simulink model "tracking_model"  (R2017a)
(part 9 of 14)

s(x_3).^4.*3.79080679921875e-6+sin(x_3).^4.*3.79080679921875e-6+cos(x_3).^4.*cos(x_4).^2.*6.757062187003037e-11+cos(x_3).^4.*cos(x_5).^2.*6.757062187003037e-11+cos(x_3).^4.*cos(x_6).^2.*6.757062187003037e-11+cos(x_3).^2.*sin(x_3).^2.*7.5816135984375e-6+cos(x_4).^2.*sin(x_3).^4.*6.757062187003037e-11+cos(x_5).^2.*sin(x_3).^4.*6.757062187003037e-11+cos(x_6).^2.*sin(x_3).^4.*6.757062187003037e-11+cos(x_3).^2.*cos(x_4).^2.*sin(x_3).^2.*1.351412437400607e-10+cos(x_3).^2.*cos(x_5).^2.*sin(x_3).^2.*1.351412437400607e-10+cos(x_3).^2.*cos(x_6).^2.*sin(x_3).^2.*1.351412437400607e-10)+(x_8.*x_9.*cos(x_3).^4.*cos(x_6).*sin(x_3).*sin(x_4).^4.*sin(x_6).*1.134624119983866e-24)./(cos(x_3).^4.*3.79080679921875e-6+sin(x_3).^4.*3.79080679921875e-6+cos(x_3).^4.*cos(x_4).^2.*6.757062187003037e-11+cos(x_3).^4.*cos(x_5).^2.*6.757062187003037e-11+cos(x_3).^4.*cos(x_6).^2.*6.757062187003037e-11+cos(x_3).^2.*sin(x_3).^2.*7.5816135984375e-6+cos(x_4).^2.*sin(x_3).^4.*6.757062187003037e-11+cos(x_5).^2.*sin(x_3).^4.*6.757062187003037e-11+cos(x_6).^2.*sin(x_3).^4.*6.757062187003037e-11+cos(x_3).^2.*cos(x_4).^2.*sin(x_3).^2.*1.351412437400607e-10+cos(x_3).^2.*cos(x_5).^2.*sin(x_3).^2.*1.351412437400607e-10+cos(x_3).^2.*cos(x_6).^2.*sin(x_3).^2.*1.351412437400607e-10)-(x_8.*x_9.*cos(x_3).*cos(x_6).*sin(x_3).^4.*sin(x_5).^4.*sin(x_6).*6.550755411017271e-25)./(cos(x_3).^4.*3.79080679921875e-6+sin(x_3).^4.*3.79080679921875e-6+cos(x_3).^4.*cos(x_4).^2.*6.757062187003037e-11+cos(x_3).^4.*cos(x_5).^2.*6.757062187003037e-11+cos(x_3).^4.*cos(x_6).^2.*6.757062187003037e-11+cos(x_3).^2.*sin(x_3).^2.*7.5816135984375e-6+cos(x_4).^2.*sin(x_3).^4.*6.757062187003037e-11+cos(x_5).^2.*sin(x_3).^4.*6.757062187003037e-11+cos(x_6).^2.*sin(x_3).^4.*6.757062187003037e-11+cos(x_3).^2.*cos(x_4).^2.*sin(x_3).^2.*1.351412437400607e-10+cos(x_3).^2.*cos(x_5).^2.*sin(x_3).^2.*1.351412437400607e-10+cos(x_3).^2.*cos(x_6).^2.*sin(x_3).^2.*1.351412437400607e-10)+(x_8.*x_9.*cos(x_3).^4.*cos(x_6).*sin(x_3).*sin(x_5).^4.*sin(x_6).*1.134624119983866e-24)./(cos(x_3).^4.*3.79080679921875e-6+sin(x_3).^4.*3.79080679921875e-6+cos(x_3).^4.*cos(x_4).^2.*6.757062187003037e-11+cos(x_3).^4.*cos(x_5).^2.*6.757062187003037e-11+cos(x_3).^4.*cos(x_6).^2.*6.757062187003037e-11+cos(x_3).^2.*sin(x_3).^2.*7.5816135984375e-6+cos(x_4).^2.*sin(x_3).^4.*6.757062187003037e-11+cos(x_5).^2.*sin(x_3).^4.*6.757062187003037e-11+cos(x_6).^2.*sin(x_3).^4.*6.757062187003037e-11+cos(x_3).^2.*cos(x_4).^2.*sin(x_3).^2.*1.351412437400607e-10+cos(x_3).^2.*cos(x_5).^2.*sin(x_3).^2.*1.351412437400607e-10+cos(x_3).^2.*cos(x_6).^2.*sin(x_3).^2.*1.351412437400607e-10)-(x_7.*x_9.*cos(x_3).*cos(x_4).*sin(x_3).^3.*sin(x_4).*sin(x_5).^2.*5.998516123203674e-18)./(cos(x_3).^4.*1.5163227196875e-5+sin(x_3).^4.*1.5163227196875e-5+cos(x_3).^4.*cos(x_4).^2.*2.702824874801215e-10+cos(x_3).^4.*cos(x_5).^2.*2.702824874801215e-10+cos(x_3).^4.*cos(x_6).^2.*2.702824874801215e-10+cos(x_3).^2.*sin(x_3).^2.*3.032645439375e-5+cos(x_4).^2.*sin(x_3).^4.*2.702824874801215e-10+cos(x_5).^2.*sin(x_3).^4.*2.702824874801215e-10+cos(x_6).^2.*sin(x_3).^4.*2.702824874801215e-10+cos(x_3).^2.*cos(x_4).^2.*sin(x_3).^2.*5.40564974960243e-10+cos(x_3).^2.*cos(x_5).^2.*sin(x_3).^2.*5.40564974960243e-10+cos(x_3).^2.*cos(x_6).^2.*sin(x_3).^2.*5.40564974960243e-10)-(x_7.*x_9.*cos(x_3).^3.*cos(x_4).*sin(x_3).*sin(x_4).*sin(x_5).^2.*5.998516123203674e-18)./(cos(x_3).^4.*1.5163227196875e-5+sin(x_3).^4.*1.5163227196875e-5+cos(x_3).^4.*cos(x_4).^2.*2.702824874801215e-10+cos(x_3).^4.*cos(x_5).^2.*2.702824874801215e-10+cos(x_3).^4.*cos(x_6).^2.*2.702824874801215e-10+cos(x_3).^2.*sin(x_3).^2.*3.032645439375e-5+cos(x_4).^2.*sin(x_3).^4.*2.702824874801215e-10+cos(x_5).^2.*sin(x_3).^4.*2.702824874801215e-10+cos(x_6).^2.*sin(x_3).^4.*2.702824874801215e-10+cos(x_3).^2.*cos(x_4).^2.*sin(x_3).^2.*5.40564974960243e-10+cos(x_3).^2.*cos(x_5).^2.*sin(x_3).^2.*5.40564974960243e-10+cos(x_3).^2.*cos(x_6).^2.*sin(x_3).^2.*5.40564974960243e-10)-(x_7.*x_9.*cos(x_3).*cos(x_4).*sin(x_3).^3.*sin(x_4).*sin(x_6).^2.*5.998516123203674e-18)./(cos(x_3).^4.*1.5163227196875e-5+sin(x_3).^4.*1.5163227196875e-5+cos(x_3).^4.*cos(x_4).^2.*2.702824874801215e-10+cos(x_3).^4.*cos(x_5).^2.*2.702824874801215e-10+cos(x_3).^4.*cos(x_6).^2.*2.702824874801215e-10+cos(x_3).^2.*sin(x_3).^2.*3.032645439375e-5+cos(x_4).^2.*sin(x_3).^4.*2.702824874801215e-10+cos(x_5).^2.*sin(x_3).^4.*2.702824874801215e-10+cos(x_6).^2.*sin(x_3).^4.*2.702824874801215e-10+cos(x_3).^2.*cos(x_4).^2.*sin(x_3).^2.*5.40564974960243e-10+cos(x_3).^2.*cos(x_5).^2.*sin(x_3).^2.*5.40564974960243e-10+cos(x_3).^2.*cos(x_6).^2.*sin(x_3).^2.*5.40564974960243e-10)+(x_7.*x_9.*cos(x_3).*cos(x_5).*sin(x_3).^3.*sin(x_4).^2.*sin(x_5).*1.607297550997493e-18)./(cos(x_3).^4.*1.5163227196875e-5+sin(x_3).^4.*1.5163227196875e-5+cos(x_3).^4.*cos(x_4).^2.*2.702824874801215e-10+cos(x_3).^4.*cos(x_5).^2.*2.702824874801215e-10+cos(x_3).^4.*cos(x_6).^2.*2.702824874801215e-10+cos(x_3).^2.*sin(x_3).^2.*3.032645439375e-5+cos(x_4).^2.*sin(x_3).^4.*2.702824874801215e-10+cos(x_5).^2.*sin(x_3).^4.*2.702824874801215e-10+cos(x_6).^2.*sin(x_3).^4.*2.702824874801215e-10+cos(x_3).^2.*cos(x_4).^2.*sin(x_3).^2.*5.40564974960243e-10+cos(x_3).^2.*cos(x_5).^2.*sin(x_3).^2.*5.40564974960243e-10+cos(x_3).^2.*cos(x_6).^2.*sin(x_3).^2.*5.40564974960243e-10)-(x_7.*x_9.*cos(x_3).^3.*cos(x_4).*sin(x_3).*sin(x_4).*sin(x_6).^2.*5.998516123203674e-18)./(cos(x_3).^4.*1.5163227196875e-5+sin(x_3).^4.*1.5163227196875e-5+cos(x_3).^4.*cos(x_4).^2.*2.702824874801215e-10+cos(x_3).^4.*cos(x_5).^2.*2.702824874801215e-10+cos(x_3).^4.*cos(x_6).^2.*2.702824874801215e-10+cos(x_3).^2.*sin(x_3).^2.*3.032645439375e-5+cos(x_4).^2.*sin(x_3).^4.*2.702824874801215e-10+cos(x_5).^2.*sin(x_3).^4.*2.702824874801215e-10+cos(x_6).^2.*sin(x_3).^4.*2.702824874801215e-10+cos(x_3).^2.*cos(x_4).^2.*sin(x_3).^2.*5.40564974960243e-10+cos(x_3).^2.*cos(x_5).^2.*sin(x_3).^2.*5.40564974960243e-10+cos(x_3).^2.*cos(x_6).^2.*sin(x_3).^2.*5.40564974960243e-10)+(x_7.*x_9.*cos(x_3).^3.*cos(x_5).*sin(x_3).*sin(x_4).^2.*sin(x_5).*1.607297550997493e-18)./(cos(x_3).^4.*1.5163227196875e-5+sin(x_3).^4.*1.5163227196875e-5+cos(x_3).^4.*cos(x_4).^2.*2.702824874801215e-10+cos(x_3).^4.*cos(x_5).^2.*2.702824874801215e-10+cos(x_3).^4.*cos(x_6).^2.*2.702824874801215e-10+cos(x_3).^2.*sin(x_3).^2.*3.032645439375e-5+cos(x_4).^2.*sin(x_3).^4.*2.702824874801215e-10+cos(x_5).^2.*sin(x_3).^4.*2.702824874801215e-10+cos(x_6).^2.*sin(x_3).^4.*2.702824874801215e-10+cos(x_3).^2.*cos(x_4).^2.*sin(x_3).^2.*5.40564974960243e-10+cos(x_3).^2.*cos(x_5).^2.*sin(x_3).^2.*5.40564974960243e-10+cos(x_3).^2.*cos(x_6).^2.*sin(x_3).^2.*5.40564974960243e-10)+(x_8.*x_9.*cos(x_3).*cos(x_4).*sin(x_3).^3.*sin(x_4).*sin(x_5).^2.*1.607297550997493e-18)./(cos(x_3).^4.*1.5163227196875e-5+sin(x_3).^4.*1.5163227196875e-5+cos(x_3).^4.*cos(x_4).^2.*2.702824874801215e-10+cos(x_3).^4.*cos(x_5).^2.*2.702824874801215e-10+cos(x_3).^4.*cos(x_6).^2.*2.702824874801215e-10+cos(x_3).^2.*sin(x_3).^2.*3.032645439375e-5+cos(x_4).^2.*sin(x_3).^4.*2.702824874801215e-10+cos(x_5).^2.*sin(x_3).^4.*2.702824874801215e-10+cos(x_6).^2.*sin(x_3).^4.*2.702824874801215e-10+cos(x_3).^2.*cos(x_4).^2.*sin(x_3).^2.*5.40564974960243e-10+cos(x_3).^2.*cos(x_5).^2.*sin(x_3).^2.*5.40564974960243e-10+cos(x_3).^2.*cos(x_6).^2.*sin(x_3).^2.*5.40564974960243e-10)+(x_8.*x_9.*cos(x_3).^3.*cos(x_4).*sin(x_3).*sin(x_4).*sin(x_5).^2.*1.607297550997493e-18)./(cos(x_3).^4.*1.5163227196875e-5+sin(x_3).^4.*1.5163227196875e-5+cos(x_3).^4.*cos(x_4).^2.*2.702824874801215e-10+cos(x_3).^4.*cos(x_5).^2.*2.702824874801215e-10+cos(x_3).^4.*cos(x_6).^2.*2.702824874801215e-10+cos(x_3).^2.*sin(x_3).^2.*3.032645439375e-5+cos(x_4).^2.*sin(x_3).^4.*2.702824874801215e-10+cos(x_5).^2.*sin(x_3).^4.*2.702824874801215e-10+cos(x_6).^2.*sin(x_3).^4.*2.702824874801215e-10+cos(x_3).^2.*cos(x_4).^2.*sin(x_3).^2.*5.40564974960243e-10+cos(x_3).^2.*cos(x_5).^2.*sin(x_3).^2.*5.40564974960243e-10+cos(x_3).^2.*cos(x_6).^2.*sin(x_3).^2.*5.40564974960243e-10)+(x_8.*x_9.*cos(x_3).*cos(x_4).*sin(x_3).^3.*sin(x_4).*sin(x_6).^2.*1.607297550997493e-18)./(cos(x_3).^4.*1.5163227196875e-5+sin(x_3).^4.*1.5163227196875e-5+cos(x_3).^4.*cos(x_4).^2.*2.702824874801215e-10+cos(x_3).^4.*cos(x_5).^2.*2.702824874801215e-10+cos(x_3).^4.*cos(x_6).^2.*2.702824874801215e-10+cos(x_3).^2.*sin(x_3).^2.*3.032645439375e-5+cos(x_4).^2.*sin(x_3).^4.*2.702824874801215e-10+cos(x_5).^2.*sin(x_3).^4.*2.702824874801215e-10+cos(x_6).^2.*sin(x_3).^4.*2.702824874801215e-10+cos(x_3).^2.*cos(x_4).^2.*sin(x_3).^2.*5.40564974960243e-10+cos(x_3).^2.*cos(x_5).^2.*sin(x_3).^2.*5.40564974960243e-10+cos(x_3).^2.*cos(x_6).^2.*sin(x_3).^2.*5.40564974960243e-10)-(x_8.*x_9.*cos(x_3).*cos(x_5).*sin(x_3).^3.*sin(x_4).^2.*sin(x_5).*5.998516123203674e-18)./(cos(x_3).^4.*1.5163227196875e-5+sin(x_3).^4.*1.5163227196875e-5+cos(x_3).^4.*cos(x_4).^2.*2.702824874801215e-10+cos(x_3).^4.*cos(x_5).^2.*2.702824874801215e-10+cos(x_3).^4.*cos(x_6).^2.*2.702824874801215e-10+cos(x_3).^2.*sin(x_3).^2.*3.032645439375e-5+cos(x_4).^2.*sin(x_3).^4.*2.702824874801215e-10+cos(x_5).^2.*sin(x_3).^4.*2.702824874801215e-10+cos(x_6).^2.*sin(x_3).^4.*2.702824874801215e-10+cos(x_3).^2.*cos(x_4).^2.*sin(x_3).^2.*5.40564974960243e-10+cos(x_3).^2.*cos(x_5).^2.*sin(x_3).^2.*5.40564974960243e-10+cos(x_3).^2.*cos(x_6).^2.*sin(x_3).^2.*5.40564974960243e-10)+(x_8.*x_9.*cos(x_3).^3.*cos(x_4).*sin(x_3).*sin(x_4).*sin(x_6).^2.*1.607297550997493e-18)./(cos(x_3).^4.*1.5163227196875e-5+sin(x_3).^4.*1.5163227196875e-5+cos(x_3).^4.*cos(x_4).^2.*2.702824874801215e-10+cos(x_3).^4.*cos(x_5).^2.*2.702824874801215e-10+cos(x_3).^4.*cos(x_6).^2.*2.702824874801215e-10+cos(x_3).^2.*sin(x_3).^2.*3.032645439375e-5+cos(x_4).^2.*sin(x_3).^4.*2.702824874801215e-10+cos(x_5).^2.*sin(x_3).^4.*2.702824874801215e-10+cos(x_6).^2.*sin(x_3).^4.*2.702824874801215e-10+cos(x_3).^2.*cos(x_4).^2.*sin(x_3).^2.*5.40564974960243e-10+cos(x_3).^2.*cos(x_5).^2.*sin(x_3).^2.*5.40564974960243e-10+cos(x_3).^2.*cos(x_6).^2.*sin(x_3).^2.*5.40564974960243e-10)-(x_8.*x_9.*cos(x_3).^3.*cos(x_5).*sin(x_3).*sin(x_4).^2.*sin(x_5).*5.998516123203674e-18)./(cos(x_3).^4.*1.5163227196875e-5+sin(x_3).^4.*1.5163227196875e-5+cos(x_3).^4.*cos(x_4).^2.*2.702824874801215e-10+cos(x_3).^4.*cos(x_5).^2.*2.702824874801215e-10+cos(x_3).^4.*cos(x_6).^2.*2.702824874801215e-10+cos(x_3).^2.*sin(x_3).^2.*3.032645439375e-5+cos(x_4).^2.*sin(x_3).^4.*2.702824874801215e-10+cos(x_5).^2.*sin(x_3).^4.*2.702824874801215e-10+cos(x_6).^2.*sin(x_3).^4.*2.702824874801215e-10+cos(x_3).^2.*cos(x_4).^2.*sin(x_3).^2.*5.40564974960243e-10+cos(x_3).^2.*cos(x_5).^2.*sin(x_3).^2.*5.40564974960243e-10+cos(x_3).^2.*cos(x_6).^2.*sin(x_3).^2.*5.40564974960243e-10)+(x_7.*x_9.*cos(x_3).*cos(x_5).*sin(x_3).^3.*sin(x_5).*sin(x_6).^2.*1.607297550997493e-18)./(cos(x_3).^4.*1.5163227196875e-5+sin(x_3).^4.*1.5163227196875e-5+cos(x_3).^4.*cos(x_4).^2.*2.702824874801215e-10+cos(x_3).^4.*cos(x_5).^2.*2.702824874801215e-10+cos(x_3).^4.*cos(x_6).^2.*2.702824874801215e-10+cos(x_3).^2.*sin(x_3).^2.*3.032645439375e-5+cos(x_4).^2.*sin(x_3).^4.*2.702824874801215e-10+cos(x_5).^2.*sin(x_3).^4.*2.702824874801215e-10+cos(x_6).^2.*sin(x_3).^4.*2.702824874801215e-10+cos(x_3).^2.*cos(x_4).^2.*sin(x_3).^2.*5.40564974960243e-10+cos(x_3).^2.*cos(x_5).^2.*sin(x_3).^2.*5.40564974960243e-10+cos(x_3).^2.*cos(x_6).^2.*sin(x_3).^2.*5.40564974960243e-10)+(x_7.*x_9.*cos(x_3).*cos(x_6).*sin(x_3).^3.*sin(x_4).^2.*sin(x_6).*4.39121857220618e-18)./(cos(x_3).^4.*1.5163227196875e-5+sin(x_3).^4.*1.5163227196875e-5+cos(x_3).^4.*cos(x_4).^2.*2.702824874801215e-10+cos(x_3).^4.*cos(x_5).^2.*2.702824874801215e-10+cos(x_3).^4.*cos(x_6).^2.*2.702824874801215e-10+cos(x_3).^2.*sin(x_3).^2.*3.032645439375e-5+cos(x_4).^2.*sin(x_3).^4.*2.702824874801215e-10+cos(x_5).^2.*sin(x_3).^4.*2.702824874801215e-10+cos(x_6).^2.*sin(x_3).^4.*2.702824874801215e-10+cos(x_3).^2.*cos(x_4).^2.*sin(x_3).^2.*5.40564974960243e-10+cos(x_3).^2.*cos(x_5).^2.*sin(x_3).^2.*5.40564974960243e-10+cos(x_3).^2.*cos(x_6).^2.*sin(x_3).^2.*5.40564974960243e-10)+(x_7.*x_9.*cos(x_3).^3.*cos(x_5).*sin(x_3).*sin(x_5).*sin(x_6).^2.*1.607297550997493e-18)./(cos(x_3).^4.*1.5163227196875e-5+sin(x_3).^4.*1.5163227196875e-5+cos(x_3).^4.*cos(x_4).^2.*2.702824874801215e-10+cos(x_3).^4.*cos(x_5).^2.*2.702824874801215e-10+cos(x_3).^4.*cos(x_6).^2.*2.702824874801215e-10+cos(x_3).^2.*sin(x_3).^2.*3.032645439375e-5+cos(x_4).^2.*sin(x_3).^4.*2.702824874801215e-10+cos(x_5).^2.*sin(x_3).^4.*2.702824874801215e-10+cos(x_6).^2.*sin(x_3).^4.*2.702824874801215e-10+cos(x_3).^2.*cos(x_4).^2.*sin(x_3).^2.*5.40564974960243e-10+cos(x_3).^2.*cos(x_5).^2.*sin(x_3).^2.*5.40564974960243e-10+cos(x_3).^2.*cos(x_6).^2.*sin(x_3).^2.*5.40564974960243e-10)+(x_7.*x_9.*cos(x_3).^3.*cos(x_6).*sin(x_3).*sin(x_4).^2.*sin(x_6).*4.39121857220618e-18)./(cos(x_3).^4.*1.5163227196875e-5+sin(x_3).^4.*1.5163227196875e-5+cos(x_3).^4.*cos(x_4).^2.*2.702824874801215e-10+cos(x_3).^4.*cos(x_5).^2.*2.702824874801215e-10+cos(x_3).^4.*cos(x_6).^2.*2.702824874801215e-10+cos(x_3).^2.*sin(x_3).^2.*3.032645439375e-5+cos(x_4).^2.*sin(x_3).^4.*2.702824874801215e-10+cos(x_5).^2.*sin(x_3).^4.*2.702824874801215e-10+cos(x_6).^2.*sin(x_3).^4.*2.702824874801215e-10+cos(x_3).^2.*cos(x_4).^2.*sin(x_3).^2.*5.40564974960243e-10+cos(x_3).^2.*cos(x_5).^2.*sin(x_3).^2.*5.40564974960243e-10+cos(x_3).^2.*cos(x_6).^2.*sin(x_3).^2.*5.40564974960243e-10)+(x_7.*x_9.*cos(x_3).*cos(x_6).*sin(x_3).^3.*sin(x_5).^2.*sin(x_6).*4.39121857220618e-18)./(cos(x_3).^4.*1.5163227196875e-5+sin(x_3).^4.*1.5163227196875e-5+cos(x_3).^4.*cos(x_4).^2.*2.702824874801215e-10+cos(x_3).^4.*cos(x_5).^2.*2.702824874801215e-10+cos(x_3).^4.*cos(x_6).^2.*2.702824874801215e-10+cos(x_3).^2.*sin(x_3).^2.*3.032645439375e-5+cos(x_4).^2.*sin(x_3).^4.*2.702824874801215e-10+cos(x_5).^2.*sin(x_3).^4.*2.702824874801215e-10+cos(x_6).^2.*sin(x_3).^4.*2.702824874801215e-10+cos(x_3).^2.*cos(x_4).^2.*sin(x_3).^2.*5.40564974960243e-10+cos(x_3).^2.*cos(x_5).^2.*sin(x_3).^2.*5.40564974960243e-10+cos(x_3).^2.*cos(x_6).^2.*sin(x_3).^2.*5.40564974960243e-10)+(x_7.*x_9.*cos(x_3).^3.*cos(x_6).*sin(x_3).*sin(x_5).^2.*sin(x_6).*4.39121857220618e-18)./(cos(x_3).^4.*1.5163227196875e-5+sin(x_3).^4.*1.5163227196875e-5+cos(x_3).^4.*cos(x_4).^2.*2.702824874801215e-10+cos(x_3).^4.*cos(x_5).^2.*2.702824874801215e-10+cos(x_3).^4.*cos(x_6).^2.*2.702824874801215e-10+cos(x_3).^2.*sin(x_3).^2.*3.032645439375e-5+cos(x_4).^2.*sin(x_3).^4.*2.702824874801215e-10+cos(x_5).^2.*sin(x_3).^4.*2.702824874801215e-10+cos(x_6).^2.*sin(x_3).^4.*2.702824874801215e-10+cos(x_3).^2.*cos(x_4).^2.*sin(x_3).^2.*5.40564974960243e-10+cos(x_3).^2.*cos(x_5).^2.*sin(x_3).^2.*5.40564974960243e-10+cos(x_3).^2.*cos(x_6).^2.*sin(x_3).^2.*5.40564974960243e-10)-(x_8.*x_9.*cos(x_3).*cos(x_5).*sin(x_3).^3.*sin(x_5).*sin(x_6).^2.*5.998516123203674e-18)./(cos(x_3).^4.*1.5163227196875e-5+sin(x_3).^4.*1.5163227196875e-5+cos(x_3).^4.*cos(x_4).^2.*2.702824874801215e-10+cos(x_3).^4.*cos(x_5).^2.*2.702824874801215e-10+cos(x_3).^4.*cos(x_6).^2.*2.702824874801215e-10+cos(x_3).^2.*sin(x_3).^2.*3.032645439375e-5+cos(x_4).^2.*sin(x_3).^4.*2.702824874801215e-10+cos(x_5).^2.*sin(x_3).^4.*2.702824874801215e-10+cos(x_6).^2.*sin(x_3).^4.*2.702824874801215e-10+cos(x_3).^2.*cos(x_4).^2.*sin(x_3).^2.*5.40564974960243e-10+cos(x_3).^2.*cos(x_5).^2.*sin(x_3).^2.*5.40564974960243e-10+cos(x_3).^2.*cos(x_6).^2.*sin(x_3).^2.*5.40564974960243e-10)+(x_8.*x_9.*cos(x_3).*cos(x_6).*sin(x_3).^3.*sin(x_4).^2.*sin(x_6).*4.39121857220618e-18)./(cos(x_3).^4.*1.5163227196875e-5+sin(x_3).^4.*1.5163227196875e-5+cos(x_3).^4.*cos(x_4).^2.*2.702824874801215e-10+cos(x_3).^4.*cos(x_5).^2.*2.702824874801215e-10+cos(x_3).^4.*cos(x_6).^2.*2.702824874801215e-10+cos(x_3).^2.*sin(x_3).^2.*3.032645439375e-5+cos(x_4).^2.*sin(x_3).^4.*2.702824874801215e-10+cos(x_5).^2.*sin(x_3).^4.*2.702824874801215e-10+cos(x_6).^2.*sin(x_3).^4.*2.702824874801215e-10+cos(x_3).^2.*cos(x_4).^2.*sin(x_3).^2.*5.40564974960243e-10+cos(x_3).^2.*cos(x_5).^2.*sin(x_3).^2.*5.40564974960243e-10+cos(x_3).^2.*cos(x_6).^2.*sin(x_3).^2.*5.40564974960243e-10)-(x_8.*x_9.*cos(x_3).^3.*cos(x_5).*sin(x_3).*sin(x_5).*sin(x_6).^2.*5.998516123203674e-18)./(cos(x_3).^4.*1.5163227196875e-5+sin(x_3).^4.*1.5163227196875e-5+cos(x_3).^4.*cos(x_4).^2.*2.702824874801215e-10+cos(x_3).^4.*cos(x_5).^2.*2.702824874801215e-10+cos(x_3).^4.*cos(x_6).^2.*2.702824874801215e-10+cos(x_3).^2.*sin(x_3).^2.*3.032645439375e-5+cos(x_4).^2.*sin(x_3).^4.*2.702824874801215e-10+cos(x_5).^2.*sin(x_3).^4.*2.702824874801215e-10+cos(x_6).^2.*sin(x_3).^4.*2.702824874801215e-10+cos(x_3).^2.*cos(x_4).^2.*sin(x_3).^2.*5.40564974960243e-10+cos(x_3).^2.*cos(x_5).^2.*sin(x_3).^2.*5.40564974960243e-10+cos(x_3).^2.*cos(x_6).^2.*sin(x_3).^2.*5.40564974960243e-10)+(x_8.*x_9.*cos(x_3).^3.*cos(x_6).*sin(x_3).*sin(x_4).^2.*sin(x_6).*4.39121857220618e-18)./(cos(x_3).^4.*1.5163227196875e-5+sin(x_3).^4.*1.5163227196875e-5+cos(x_3).^4.*cos(x_4).^2.*2.702824874801215e-10+cos(x_3).^4.*cos(x_5).^2.*2.702824874801215e-10+cos(x_3).^4.*cos(x_6).^2.*2.702824874801215e-10+cos(x_3).^2.*sin(x_3).^2.*3.032645439375e-5+cos(x_4).^2.*sin(x_3).^4.*2.702824874801215e-10+cos(x_5).^2.*sin(x_3).^4.*2.702824874801215e-10+cos(x_6).^2.*sin(x_3).^4.*2.702824874801215e-10+cos(x_3).^2.*cos(x_4).^2.*sin(x_3).^2.*5.40564974960243e-10+cos(x_3).^2.*cos(x_5).^2.*sin(x_3).^2.*5.40564974960243e-10+cos(x_3).^2.*cos(x_6).^2.*sin(x_3).^2.*5.40564974960243e-10)+(x_8.*x_9.*cos(x_3).*cos(x_6).*sin(x_3).^3.*sin(x_5).^2.*sin(x_6).*4.39121857220618e-18)./(cos(x_3).^4.*1.5163227196875e-5+sin(x_3).^4.*1.5163227196875e-5+cos(x_3).^4.*cos(x_4).^2.*2.702824874801215e-10+cos(x_3).^4.*cos(x_5).^2.*2.702824874801215e-10+cos(x_3).^4.*cos(x_6).^2.*2.702824874801215e-10+cos(x_3).^2.*sin(x_3).^2.*3.032645439375e-5+cos(x_4).^2.*sin(x_3).^4.*2.702824874801215e-10+cos(x_5).^2.*sin(x_3).^4.*2.702824874801215e-10+cos(x_6).^2.*sin(x_3).^4.*2.702824874801215e-10+cos(x_3).^2.*cos(x_4).^2.*sin(x_3).^2.*5.40564974960243e-10+cos(x_3).^2.*cos(x_5).^2.*sin(x_3).^2.*5.40564974960243e-10+cos(x_3).^2.*cos(x_6).^2.*sin(x_3).^2.*5.40564974960243e-10)+(x_8.*x_9.*cos(x_3).^3.*cos(x_6).*sin(x_3).*sin(x_5).^2.*sin(x_6).*4.39121857220618e-18)./(cos(x_3).^4.*1.5163227196875e-5+sin(x_3).^4.*1.5163227196875e-5+cos(x_3).^4.*cos(x_4).^2.*2.702824874801215e-10+cos(x_3).^4.*cos(x_5).^2.*2.702824874801215e-10+cos(x_3).^4.*cos(x_6).^2.*2.702824874801215e-10+cos(x_3).^2.*sin(x_3).^2.*3.032645439375e-5+cos(x_4).^2.*sin(x_3).^4.*2.702824874801215e-10+cos(x_5).^2.*sin(x_3).^4.*2.702824874801215e-10+cos(x_6).^2.*sin(x_3).^4.*2.702824874801215e-10+cos(x_3).^2.*cos(x_4).^2.*sin(x_3).^2.*5.40564974960243e-10+cos(x_3).^2.*cos(x_5).^2.*sin(x_3).^2.*5.40564974960243e-10+cos(x_3).^2.*cos(x_6).^2.*sin(x_3).^2.*5.40564974960243e-10)+(x_7.*x_9.*cos(x_3).^2.*cos(x_4).*sin(x_3).^3.*sin(x_4).*sin(x_5).^2.*2.94020985815061e-19)./(cos(x_3).^4.*3.79080679921875e-6+sin(x_3).^4.*3.79080679921875e-6+cos(x_3).^4.*cos(x_4).^2.*6.757062187003037e-11+cos(x_3).^4.*cos(x_5).^2.*6.757062187003037e-11+cos(x_3).^4.*cos(x_6).^2.*6.757062187003037e-11+cos(x_3).^2.*sin(x_3).^2.*7.5816135984375e-6+cos(x_4).^2.*sin(x_3).^4.*6.757062187003037e-11+cos(x_5).^2.*sin(x_3).^4.*6.757062187003037e-11+cos(x_6).^2.*sin(x_3).^4.*6.757062187003037e-11+cos(x_3).^2.*cos(x_4).^2.*sin(x_3).^2.*1.351412437400607e-10+cos(x_3).^2.*cos(x_5).^2.*sin(x_3).^2.*1.351412437400607e-10+cos(x_3).^2.*cos(x_6).^2.*sin(x_3).^2.*1.351412437400607e-10)+(x_7.*x_9.*cos(x_3).^2.*cos(x_4).*sin(x_3).^3.*sin(x_4).*sin(x_6).^2.*2.94020985815061e-19)./(cos(x_3).^4.*3.79080679921875e-6+sin(x_3).^4.*3.79080679921875e-6+cos(x_3).^4.*cos(x_4).^2.*6.757062187003037e-11+cos(x_3).^4.*cos(x_5).^2.*6.757062187003037e-11+cos(x_3).^4.*cos(x_6).^2.*6.757062187003037e-11+cos(x_3).^2.*sin(x_3).^2.*7.5816135984375e-6+cos(x_4).^2.*sin(x_3).^4.*6.757062187003037e-11+cos(x_5).^2.*sin(x_3).^4.*6.757062187003037e-11+cos(x_6).^2.*sin(x_3).^4.*6.757062187003037e-11+cos(x_3).^2.*cos(x_4).^2.*sin(x_3).^2.*1.351412437400607e-10+cos(x_3).^2.*cos(x_5).^2.*sin(x_3).^2.*1.351412437400607e-10+cos(x_3).^2.*cos(x_6).^2.*sin(x_3).^2.*1.351412437400607e-10)-(x_7.*x_9.*cos(x_3).^2.*cos(x_5).*sin(x_3).^3.*sin(x_4).^2.*sin(x_5).*1.470104929075305e-19)./(cos(x_3).^4.*3.79080679921875e-6+sin(x_3).^4.*3.79080679921875e-6+cos(x_3).^4.*cos(x_4).^2.*6.757062187003037e-11+cos(x_3).^4.*cos(x_5).^2.*6.757062187003037e-11+cos(x_3).^4.*cos(x_6).^2.*6.757062187003037e-11+cos(x_3).^2.*sin(x_3).^2.*7.5816135984375e-6+cos(x_4).^2.*sin(x_3).^4.*6.757062187003037e-11+cos(x_5).^2.*sin(x_3).^4.*6.757062187003037e-11+cos(x_6).^2.*sin(x_3).^4.*6.757062187003037e-11+cos(x_3).^2.*cos(x_4).^2.*sin(x_3).^2.*1.351412437400607e-10+cos(x_3).^2.*cos(x_5).^2.*sin(x_3).^2.*1.351412437400607e-10+cos(x_3).^2.*cos(x_6).^2.*sin(x_3).^2.*1.351412437400607e-10)+(x_7.*x_9.*cos(x_3).^3.*cos(x_5).*sin(x_3).^2.*sin(x_4).^2.*sin(x_5).*2.546296429615869e-19)./(cos(x_3).^4.*3.79080679921875e-6+sin(x_3).^4.*3.79080679921875e-6+cos(x_3).^4.*cos(x_4).^2.*6.757062187003037e-11+cos(x_3).^4.*cos(x_5).^2.*6.757062187003037e-11+cos(x_3).^4.*cos(x_6).^2.*6.757062187003037e-11+cos(x_3).^2.*sin(x_3).^2.*7.5816135984375e-6+cos(x_4).^2.*sin(x_3).^4.*6.757062187003037e-11+cos(x_5).^2.*sin(x_3).^4.*6.757062187003037e-11+cos(x_6).^2.*sin(x_3).^4.*6.757062187003037e-11+cos(x_3).^2.*cos(x_4).^2.*sin(x_3).^2.*1.351412437400607e-10+cos(x_3).^2.*cos(x_5).^2.*sin(x_3).^2.*1.351412437400607e-10+cos(x_3).^2.*cos(x_6).^2.*sin(x_3).^2.*1.351412437400607e-10)-(x_8.*x_9.*cos(x_3).^3.*cos(x_4).*sin(x_3).^2.*sin(x_4).*sin(x_5).^2.*2.94020985815061e-19)./(cos(x_3).^4.*3.79080679921875e-6+sin(x_3).^4.*3.79080679921875e-6+cos(x_3).^4.*cos(x_4).^2.*6.757062187003037e-11+cos(x_3).^4.*cos(x_5).^2.*6.757062187003037e-11+cos(x_3).^4.*cos(x_6).^2.*6.757062187003037e-11+cos(x_3).^2.*sin(x_3).^2.*7.5816135984375e-6+cos(x_4).^2.*sin(x_3).^4.*6.757062187003037e-11+cos(x_5).^2.*sin(x_3).^4.*6.757062187003037e-11+cos(x_6).^2.*sin(x_3).^4.*6.757062187003037e-11+cos(x_3).^2.*cos(x_4).^2.*sin(x_3).^2.*1.351412437400607e-10+cos(x_3).^2.*cos(x_5).^2.*sin(x_3).^2.*1.351412437400607e-10+cos(x_3).^2.*cos(x_6).^2.*sin(x_3).^2.*1.351412437400607e-10)-(x_7.*x_9.*cos(x_3).^2.*cos(x_4).*sin(x_3).^3.*sin(x_4).*sin(x_5).^4.*2.620302164406908e-24)./(cos(x_3).^4.*3.79080679921875e-6+sin(x_3).^4.*3.79080679921875e-6+cos(x_3).^4.*cos(x_4).^2.*6.757062187003037e-11+cos(x_3).^4.*cos(x_5).^2.*6.757062187003037e-11+cos(x_3).^4.*cos(x_6).^2.*6.757062187003037e-11+cos(x_3).^2.*sin(x_3).^2.*7.5816135984375e-6+cos(x_4).^2.*sin(x_3).^4.*6.757062187003037e-11+cos(x_5).^2.*sin(x_3).^4.*6.757062187003037e-11+cos(x_6).^2.*sin(x_3).^4.*6.757062187003037e-11+cos(x_3).^2.*cos(x_4).^2.*sin(x_3).^2.*1.351412437400607e-10+cos(x_3).^2.*cos(x_5).^2.*sin(x_3).^2.*1.351412437400607e-10+cos(x_3).^2.*cos(x_6).^2.*sin(x_3).^2.*1.351412437400607e-10)-(x_7.*x_9.*cos(x_3).^4.*cos(x_4).*sin(x_3).*sin(x_4).^3.*sin(x_5).^2.*2.620302164406908e-24)./(cos(x_3).^4.*3.79080679921875e-6+sin(x_3).^4.*3.79080679921875e-6+cos(x_3).^4.*cos(x_4).^2.*6.757062187003037e-11+cos(x_3).^4.*cos(x_5).^2.*6.757062187003037e-11+cos(x_3).^4.*cos(x_6).^2.*6.757062187003037e-11+cos(x_3).^2.*sin(x_3).^2.*7.5816135984375e-6+cos(x_4).^2.*sin(x_3).^4.*6.757062187003037e-11+cos(x_5).^2.*sin(x_3).^4.*6.757062187003037e-11+cos(x_6).^2.*sin(x_3).^4.*6.757062187003037e-11+cos(x_3).^2.*cos(x_4).^2.*sin(x_3).^2.*1.351412437400607e-10+cos(x_3).^2.*cos(x_5).^2.*sin(x_3).^2.*1.351412437400607e-10+cos(x_3).^2.*cos(x_6).^2.*sin(x_3).^2.*1.351412437400607e-10)+(x_8.*x_9.*cos(x_3).^2.*cos(x_5).*sin(x_3).^3.*sin(x_4).^2.*sin(x_5).*2.546296429615869e-19)./(cos(x_3).^4.*3.79080679921875e-6+sin(x_3).^4.*3.79080679921875e-6+cos(x_3).^4.*cos(x_4).^2.*6.757062187003037e-11+cos(x_3).^4.*cos(x_5).^2.*6.757062187003037e-11+cos(x_3).^4.*cos(x_6).^2.*6.757062187003037e-11+cos(x_3).^2.*sin(x_3).^2.*7.5816135984375e-6+cos(x_4).^2.*sin(x_3).^4.*6.757062187003037e-11+cos(x_5).^2.*sin(x_3).^4.*6.757062187003037e-11+cos(x_6).^2.*sin(x_3).^4.*6.757062187003037e-11+cos(x_3).^2.*cos(x_4).^2.*sin(x_3).^2.*1.351412437400607e-10+cos(x_3).^2.*cos(x_5).^2.*sin(x_3).^2.*1.351412437400607e-10+cos(x_3).^2.*cos(x_6).^2.*sin(x_3).^2.*1.351412437400607e-10)-(x_8.*x_9.*cos(x_3).^3.*cos(x_4).*sin(x_3).^2.*sin(x_4).*sin(x_6).^2.*2.94020985815061e-19)./(cos(x_3).^4.*3.79080679921875e-6+sin(x_3).^4.*3.79080679921875e-6+cos(x_3).^4.*cos(x_4).^2.*6.757062187003037e-11+cos(x_3).^4.*cos(x_5).^2.*6.757062187003037e-11+cos(x_3).^4.*cos(x_6).^2.*6.757062187003037e-11+cos(x_3).^2.*sin(x_3).^2.*7.5816135984375e-6+cos(x_4).^2.*sin(x_3).^4.*6.757062187003037e-11+cos(x_5).^2.*sin(x_3).^4.*6.757062187003037e-11+cos(x_6).^2.*sin(x_3).^4.*6.757062187003037e-11+cos(x_3).^2.*cos(x_4).^2.*sin(x_3).^2.*1.351412437400607e-10+cos(x_3).^2.*cos(x_5).^2.*sin(x_3).^2.*1.351412437400607e-10+cos(x_3).^2.*cos(x_6).^2.*sin(x_3).^2.*1.351412437400607e-10)+(x_8.*x_9.*cos(x_3).^3.*cos(x_5).*sin(x_3).^2.*sin(x_4).^2.*sin(x_5).*1.470104929075305e-19)./(cos(x_3).^4.*3.79080679921875e-6+sin(x_3).^4.*3.79080679921875e-6+cos(x_3).^4.*cos(x_4).^2.*6.757062187003037e-11+cos(x_3).^4.*cos(x_5).^2.*6.757062187003037e-11+cos(x_3).^4.*cos(x_6).^2.*6.757062187003037e-11+cos(x_3).^2.*sin(x_3).^2.*7.5816135984375e-6+cos(x_4).^2.*sin(x_3).^4.*6.757062187003037e-11+cos(x_5).^2.*sin(x_3).^4.*6.757062187003037e-11+cos(x_6).^2.*sin(x_3).^4.*6.757062187003037e-11+cos(x_3).^2.*cos(x_4).^2.*sin(x_3).^2.*1.351412437400607e-10+cos(x_3).^2.*cos(x_5).^2.*sin(x_3).^2.*1.351412437400607e-10+cos(x_3).^2.*cos(x_6).^2.*sin(x_3).^2.*1.351412437400607e-10)-(x_7.*x_9.*cos(x_3).*cos(x_5).*sin(x_3).^4.*sin(x_4).^2.*sin(x_5).^3.*2.269248239967731e-24)./(cos(x_3).^4.*3.79080679921875e-6+sin(x_3).^4.*3.79080679921875e-6+cos(x_3).^4.*cos(x_4).^2.*6.757062187003037e-11+cos(x_3).^4.*cos(x_5).^2.*6.757062187003037e-11+cos(x_3).^4.*cos(x_6).^2.*6.757062187003037e-11+cos(x_3).^2.*sin(x_3).^2.*7.5816135984375e-6+cos(x_4).^2.*sin(x_3).^4.*6.757062187003037e-11+cos(x_5).^2.*sin(x_3).^4.*6.757062187003037e-11+cos(x_6).^2.*sin(x_3).^4.*6.757062187003037e-11+cos(x_3).^2.*cos(x_4).^2.*sin(x_3).^2.*1.351412437400607e-10+cos(x_3).^2.*cos(x_5).^2.*sin(x_3).^2.*1.351412437400607e-10+cos(x_3).^2.*cos(x_6).^2.*sin(x_3).^2.*1.351412437400607e-10)-(x_7.*x_9.*cos(x_3).^2.*cos(x_4).*sin(x_3).^3.*sin(x_4).*sin(x_6).^4.*2.620302164406908e-24)./(cos(x_3).^4.*3.79080679921875e-6+sin(x_3).^4.*3.79080679921875e-6+cos(x_3).^4.*cos(x_4).^2.*6.757062187003037e-11+cos(x_3).^4.*cos(x_5).^2.*6.757062187003037e-11+cos(x_3).^4.*cos(x_6).^2.*6.757062187003037e-11+cos(x_3).^2.*sin(x_3).^2.*7.5816135984375e-6+cos(x_4).^2.*sin(x_3).^4.*6.757062187003037e-11+cos(x_5).^2.*sin(x_3).^4.*6.757062187003037e-11+cos(x_6).^2.*sin(x_3).^4.*6.757062187003037e-11+cos(x_3).^2.*cos(x_4).^2.*sin(x_3).^2.*1.351412437400607e-10+cos(x_3).^2.*cos(x_5).^2.*sin(x_3).^2.*1.351412437400607e-10+cos(x_3).^2.*cos(x_6).^2.*sin(x_3).^2.*1.351412437400607e-10)-(x_7.*x_9.*cos(x_3).^2.*cos(x_5).*sin(x_3).^3.*sin(x_5).*sin(x_6).^2.*1.470104929075305e-19)./(cos(x_3).^4.*3.79080679921875e-6+sin(x_3).^4.*3.79080679921875e-6+cos(x_3).^4.*cos(x_4).^2.*6.757062187003037e-11+cos(x_3).^4.*cos(x_5).^2.*6.757062187003037e-11+cos(x_3).^4.*cos(x_6).^2.*6.757062187003037e-11+cos(x_3).^2.*sin(x_3).^2.*7.5816135984375e-6+cos(x_4).^2.*sin(x_3).^4.*6.757062187003037e-11+cos(x_5).^2.*sin(x_3).^4.*6.757062187003037e-11+cos(x_6).^2.*sin(x_3).^4.*6.757062187003037e-11+cos(x_3).^2.*cos(x_4).^2.*sin(x_3).^2.*1.351412437400607e-10+cos(x_3).^2.*cos(x_5).^2.*sin(x_3).^2.*1.351412437400607e-10+cos(x_3).^2.*cos(x_6).^2.*sin(x_3).^2.*1.351412437400607e-10)+(x_7.*x_9.*cos(x_3).^2.*cos(x_5).*sin(x_3).^3.*sin(x_4).^4.*sin(x_5).*1.310151082203454e-24)./(cos(x_3).^4.*3.79080679921875e-6+sin(x_3).^4.*3.79080679921875e-6+cos(x_3).^4.*cos(x_4).^2.*6.757062187003037e-11+cos(x_3).^4.*cos(x_5).^2.*6.757062187003037e-11+cos(x_3).^4.*cos(x_6).^2.*6.757062187003037e-11+cos(x_3).^2.*sin(x_3).^2.*7.5816135984375e-6+cos(x_4).^2.*sin(x_3).^4.*6.757062187003037e-11+cos(x_5).^2.*sin(x_3).^4.*6.757062187003037e-11+cos(x_6).^2.*sin(x_3).^4.*6.757062187003037e-11+cos(x_3).^2.*cos(x_4).^2.*sin(x_3).^2.*1.351412437400607e-10+cos(x_3).^2.*cos(x_5).^2.*sin(x_3).^2.*1.351412437400607e-10+cos(x_3).^2.*cos(x_6).^2.*sin(x_3).^2.*1.351412437400607e-10)-(x_7.*x_9.*cos(x_3).^2.*cos(x_6).*sin(x_3).^3.*sin(x_4).^2.*sin(x_6).*1.470104929075305e-19)./(cos(x_3).^4.*3.79080679921875e-6+sin(x_3).^4.*3.79080679921875e-6+cos(x_3).^4.*cos(x_4).^2.*6.757062187003037e-11+cos(x_3).^4.*cos(x_5).^2.*6.757062187003037e-11+cos(x_3).^4.*cos(x_6).^2.*6.757062187003037e-11+cos(x_3).^2.*sin(x_3).^2.*7.5816135984375e-6+cos(x_4).^2.*sin(x_3).^4.*6.757062187003037e-11+cos(x_5).^2.*sin(x_3).^4.*6.757062187003037e-11+cos(x_6).^2.*sin(x_3).^4.*6.757062187003037e-11+cos(x_3).^2.*cos(x_4).^2.*sin(x_3).^2.*1.351412437400607e-10+cos(x_3).^2.*cos(x_5).^2.*sin(x_3).^2.*1.351412437400607e-10+cos(x_3).^2.*cos(x_6).^2.*sin(x_3).^2.*1.351412437400607e-10)+(x_7.*x_9.*cos(x_3).^3.*cos(x_5).*sin(x_3).^2.*sin(x_5).*sin(x_6).^2.*2.546296429615869e-19)./(cos(x_3).^4.*3.79080679921875e-6+sin(x_3).^4.*3.79080679921875e-6+cos(x_3).^4.*cos(x_4).^2.*6.757062187003037e-11+cos(x_3).^4.*cos(x_5).^2.*6.757062187003037e-11+cos(x_3).^4.*cos(x_6).^2.*6.757062187003037e-11+cos(x_3).^2.*sin(x_3).^2.*7.5816135984375e-6+cos(x_4).^2.*sin(x_3).^4.*6.757062187003037e-11+cos(x_5).^2.*sin(x_3).^4.*6.757062187003037e-11+cos(x_6).^2.*sin(x_3).^4.*6.757062187003037e-11+cos(x_3).^2.*cos(x_4).^2.*sin(x_3).^2.*1.351412437400607e-10+cos(x_3).^2.*cos(x_5).^2.*sin(x_3).^2.*1.351412437400607e-10+cos(x_3).^2.*cos(x_6).^2.*sin(x_3).^2.*1.351412437400607e-10)-(x_7.*x_9.*cos(x_3).^3.*cos(x_5).*sin(x_3).^2.*sin(x_4).^4.*sin(x_5).*2.269248239967731e-24)./(cos(x_3).^4.*3.79080679921875e-6+sin(x_3).^4.*3.79080679921875e-6+cos(x_3).^4.*cos(x_4).^2.*6.757062187003037e-11+cos(x_3).^4.*cos(x_5).^2.*6.757062187003037e-11+cos(x_3).^4.*cos(x_6).^2.*6.757062187003037e-11+cos(x_3).^2.*sin(x_3).^2.*7.5816135984375e-6+cos(x_4).^2.*sin(x_3).^4.*6.757062187003037e-11+cos(x_5).^2.*sin(x_3).^4.*6.757062187003037e-11+cos(x_6).^2.*sin(x_3).^4.*6.757062187003037e-11+cos(x_3).^2.*cos(x_4).^2.*sin(x_3).^2.*1.351412437400607e-10+cos(x_3).^2.*cos(x_5).^2.*sin(x_3).^2.*1.351412437400607e-10+cos(x_3).^2.*cos(x_6).^2.*sin(x_3).^2.*1.351412437400607e-10)-(x_7.*x_9.*cos(x_3).^3.*cos(x_6).*sin(x_3).^2.*sin(x_4).^2.*sin(x_6).*2.546296429615869e-19)./(cos(x_3).^4.*3.79080679921875e-6+sin(x_3).^4.*3.79080679921875e-6+cos(x_3).^4.*cos(x_4).^2.*6.757062187003037e-11+cos(x_3).^4.*cos(x_5).^2.*6.757062187003037e-11+cos(x_3).^4.*cos(x_6).^2.*6.757062187003037e-11+cos(x_3).^2.*sin(x_3).^2.*7.5816135984375e-6+cos(x_4).^2.*sin(x_3).^4.*6.757062187003037e-11+cos(x_5).^2.*sin(x_3).^4.*6.757062187003037e-11+cos(x_6).^2.*sin(x_3).^4.*6.757062187003037e-11+cos(x_3).^2.*cos(x_4).^2.*sin(x_3).^2.*1.351412437400607e-10+cos(x_3).^2.*cos(x_5).^2.*sin(x_3).^2.*1.351412437400607e-10+cos(x_3).^2.*cos(x_6).^2.*sin(x_3).^2.*1.351412437400607e-10)-(x_7.*x_9.*cos(x_3).^4.*cos(x_4).*sin(x_3).*sin(x_4).^3.*sin(x_6).^2.*2.620302164406908e-24)./(cos(x_3).^4.*3.79080679921875e-6+sin(x_3).^4.*3.79080679921875e-6+cos(x_3).^4.*cos(x_4).^2.*6.757062187003037e-11+cos(x_3).^4.*cos(x_5).^2.*6.757062187003037e-11+cos(x_3).^4.*cos(x_6).^2.*6.757062187003037e-11+cos(x_3).^2.*sin(x_3).^2.*7.5816135984375e-6+cos(x_4).^2.*sin(x_3).^4.*6.757062187003037e-11+cos(x_5).^2.*sin(x_3).^4.*6.757062187003037e-11+cos(x_6).^2.*sin(x_3).^4.*6.757062187003037e-11+cos(x_3).^2.*cos(x_4).^2.*sin(x_3).^2.*1.351412437400607e-10+cos(x_3).^2.*cos(x_5).^2.*sin(x_3).^2.*1.351412437400607e-10+cos(x_3).^2.*cos(x_6).^2.*sin(x_3).^2.*1.351412437400607e-10)+(x_7.*x_9.*cos(x_3).^4.*cos(x_5).*sin(x_3).*sin(x_4).^2.*sin(x_5).^3.*1.310151082203454e-24)./(cos(x_3).^4.*3.79080679921875e-6+sin(x_3).^4.*3.79080679921875e-6+cos(x_3).^4.*cos(x_4).^2.*6.757062187003037e-11+cos(x_3).^4.*cos(x_5).^2.*6.757062187003037e-11+cos(x_3).^4.*cos(x_6).^2.*6.757062187003037e-11+cos(x_3).^2.*sin(x_3).^2.*7.5816135984375e-6+cos(x_4).^2.*sin(x_3).^4.*6.757062187003037e-11+cos(x_5).^2.*sin(x_3).^4.*6.757062187003037e-11+cos(x_6).^2.*sin(x_3).^4.*6.757062187003037e-11+cos(x_3).^2.*cos(x_4).^2.*sin(x_3).^2.*1.351412437400607e-10+cos(x_3).^2.*cos(x_5).^2.*sin(x_3).^2.*1.351412437400607e-10+cos(x_3).^2.*cos(x_6).^2.*sin(x_3).^2.*1.351412437400607e-10)+(x_8.*x_9.*cos(x_3).*cos(x_4).*sin(x_3).^4.*sin(x_4).^3.*sin(x_5).^2.*2.620302164406908e-24)./(cos(x_3).^4.*3.79080679921875e-6+sin(x_3).^4.*3.79080679921875e-6+cos(x_3).^4.*cos(x_4).^2.*6.757062187003037e-11+cos(x_3).^4.*cos(x_5).^2.*6.757062187003037e-11+cos(x_3).^4.*cos(x_6).^2.*6.757062187003037e-11+cos(x_3).^2.*sin(x_3).^2.*7.5816135984375e-6+cos(x_4).^2.*sin(x_3).^4.*6.757062187003037e-11+cos(x_5).^2.*sin(x_3).^4.*6.757062187003037e-11+cos(x_6).^2.*sin(x_3).^4.*6.757062187003037e-11+cos(x_3).^2.*cos(x_4).^2.*sin(x_3).^2.*1.351412437400607e-10+cos(x_3).^2.*cos(x_5).^2.*sin(x_3).^2.*1.351412437400607e-10+cos(x_3).^2.*cos(x_6).^2.*sin(x_3).^2.*1.351412437400607e-10)+(x_8.*x_9.*cos(x_3).^3.*cos(x_4).*sin(x_3).^2.*sin(x_4).*sin(x_5).^4.*2.620302164406908e-24)./(cos(x_3).^4.*3.79080679921875e-6+sin(x_3).^4.*3.79080679921875e-6+cos(x_3).^4.*cos(x_4).^2.*6.757062187003037e-11+cos(x_3).^4.*cos(x_5).^2.*6.757062187003037e-11+cos(x_3).^4.*cos(x_6).^2.*6.757062187003037e-11+cos(x_3).^2.*sin(x_3).^2.*7.5816135984375e-6+cos(x_4).^2.*sin(x_3).^4.*6.757062187003037e-11+cos(x_5).^2.*sin(x_3).^4.*6.757062187003037e-11+cos(x_6).^2.*sin(x_3).^4.*6.757062187003037e-11+cos(x_3).^2.*cos(x_4).^2.*sin(x_3).^2.*1.351412437400607e-10+cos(x_3).^2.*cos(x_5).^2.*sin(x_3).^2.*1.351412437400607e-10+cos(x_3).^2.*cos(x_6).^2.*sin(x_3).^2.*1.351412437400607e-10)-(x_7.*x_9.*cos(x_3).^2.*cos(x_6).*sin(x_3).^3.*sin(x_5).^2.*sin(x_6).*1.470104929075305e-19)./(cos(x_3).^4.*3.79080679921875e-6+sin(x_3).^4.*3.79080679921875e-6+cos(x_3).^4.*cos(x_4).^2.*6.757062187003037e-11+cos(x_3).^4.*cos(x_5).^2.*6.757062187003037e-11+cos(x_3).^4.*cos(x_6).^2.*6.757062187003037e-11+cos(x_3).^2.*sin(x_3).^2.*7.5816135984375e-6+cos(x_4).^2.*sin(x_3).^4.*6.757062187003037e-11+cos(x_5).^2.*sin(x_3).^4.*6.757062187003037e-11+cos(x_6).^2.*sin(x_3).^4.*6.757062187003037e-11+cos(x_3).^2.*cos(x_4).^2.*sin(x_3).^2.*1.351412437400607e-10+cos(x_3).^2.*cos(x_5).^2.*sin(x_3).^2.*1.351412437400607e-10+cos(x_3).^2.*cos(x_6).^2.*sin(x_3).^2.*1.351412437400607e-10)-(x_7.*x_9.*cos(x_3).^3.*cos(x_6).*sin(x_3).^2.*sin(x_5).^2.*sin(x_6).*2.546296429615869e-19)./(cos(x_3).^4.*3.79080679921875e-6+sin(x_3).^4.*3.79080679921875e-6+cos(x_3).^4.*cos(x_4).^2.*6.757062187003037e-11+cos(x_3).^4.*cos(x_5).^2.*6.757062187003037e-11+cos(x_3).^4.*cos(x_6).^2.*6.757062187003037e-11+cos(x_3).^2.*sin(x_3).^2.*7.5816135984375e-6+cos(x_4).^2.*sin(x_3).^4.*6.757062187003037e-11+cos(x_5).^2.*sin(x_3).^4.*6.757062187003037e-11+cos(x_6).^2.*sin(x_3).^4.*6.757062187003037e-11+cos(x_3).^2.*cos(x_4).^2.*sin(x_3).^2.*1.351412437400607e-10+cos(x_3).^2.*cos(x_5).^2.*sin(x_3).^2.*1.351412437400607e-10+cos(x_3).^2.*cos(x_6).^2.*sin(x_3).^2.*1.351412437400607e-10)+(x_8.*x_9.*cos(x_3).*cos(x_4).*sin(x_3).^4.*sin(x_4).^3.*sin(x_6).^2.*2.620302164406908e-24)./(cos(x_3).^4.*3.79080679921875e-6+sin(x_3).^4.*3.79080679921875e-6+cos(x_3).^4.*cos(x_4).^2.*6.757062187003037e-11+cos(x_3).^4.*cos(x_5).^2.*6.757062187003037e-11+cos(x_3).^4.*cos(x_6).^2.*6.757062187003037e-11+cos(x_3).^2.*sin(x_3).^2.*7.5816135984375e-6+cos(x_4).^2.*sin(x_3).^4.*6.757062187003037e-11+cos(x_5).^2.*sin(x_3).^4.*6.757062187003037e-11+cos(x_6).^2.*sin(x_3).^4.*6.757062187003037e-11+cos(x_3).^2.*cos(x_4).^2.*sin(x_3).^2.*1.351412437400607e-10+cos(x_3).^2.*cos(x_5).^2.*sin(x_3).^2.*1.351412437400607e-10+cos(x_3).^2.*cos(x_6).^2.*sin(x_3).^2.*1.351412437400607e-10)-(x_8.*x_9.*cos(x_3).*cos(x_5).*sin(x_3).^4.*sin(x_4).^2.*sin(x_5).^3.*1.310151082203454e-24)./(cos(x_3).^4.*3.79080679921875e-6+sin(x_3).^4.*3.79080679921875e-6+cos(x_3).^4.*cos(x_4).^2.*6.757062187003037e-11+cos(x_3).^4.*cos(x_5).^2.*6.757062187003037e-11+cos(x_3).^4.*cos(x_6).^2.*6.757062187003037e-11+cos(x_3).^2.*sin(x_3).^2.*7.5816135984375e-6+cos(x_4).^2.*sin(x_3).^4.*6.757062187003037e-11+cos(x_5).^2.*sin(x_3).^4.*6.757062187003037e-11+cos(x_6).^2.*sin(x_3).^4.*6.757062187003037e-11+cos(x_3).^2.*cos(x_4).^2.*sin(x_3).^2.*1.351412437400607e-10+cos(x_3).^2.*cos(x_5).^2.*sin(x_3).^2.*1.351412437400607e-10+cos(x_3).^2.*cos(x_6).^2.*sin(x_3).^2.*1.351412437400607e-10)+(x_8.*x_9.*cos(x_3).^2.*cos(x_5).*sin(x_3).^3.*sin(x_5).*sin(x_6).^2.*2.546296429615869e-19)./(cos(x_3).^4.*3.79080679921875e-6+sin(x_3).^4.*3.79080679921875e-6+cos(x_3).^4.*cos(x_4).^2.*6.757062187003037e-11+cos(x_3).^4.*cos(x_5).^2.*6.757062187003037e-11+cos(x_3).^4.*cos(x_6).^2.*6.757062187003037e-11+cos(x_3).^2.*sin(x_3).^2.*7.5816135984375e-6+cos(x_4).^2.*sin(x_3).^4.*6.757062187003037e-11+cos(x_5).^2.*sin(x_3).^4.*6.757062187003037e-11+cos(x_6).^2.*sin(x_3).^4.*6.757062187003037e-11+cos(x_3).^2.*cos(x_4).^2.*sin(x_3).^2.*1.351412437400607e-10+cos(x_3).^2.*cos(x_5).^2.*sin(x_3).^2.*1.351412437400607e-10+cos(x_3).^2.*cos(x_6).^2.*sin(x_3).^2.*1.351412437400607e-10)-(x_8.*x_9.*cos(x_3).^2.*cos(x_5).*sin(x_3).^3.*sin(x_4).^4.*sin(x_5).*2.269248239967731e-24)./(cos(x_3).^4.*3.79080679921875e-6+sin(x_3).^4.*3.79080679921875e-6+cos(x_3).^4.*cos(x_4).^2.*6.757062187003037e-11+cos(x_3).^4.*cos(x_5).^2.*6.757062187003037e-11+cos(x_3).^4.*cos(x_6).^2.*6.757062187003037e-11+cos(x_3).^2.*sin(x_3).^2.*7.5816135984375e-6+cos(x_4).^2.*sin(x_3).^4.*6.757062187003037e-11+cos(x_5).^2.*sin(x_3).^4.*6.757062187003037e-11+cos(x_6).^2.*sin(x_3).^4.*6.757062187003037e-11+cos(x_3).^2.*cos(x_4).^2.*sin(x_3).^2.*1.351412437400607e-10+cos(x_3).^2.*cos(x_5).^2.*sin(x_3).^2.*1.351412437400607e-10+cos(x_3).^2.*cos(x_6).^2.*sin(x_3).^2.*1.351412437400607e-10)-(x_8.*x_9.*cos(x_3).^2.*cos(x_6).*sin(x_3).^3.*sin(x_4).^2.*sin(x_6).*2.546296429615869e-19)./(cos(x_3).^4.*3.79080679921875e-6+sin(x_3).^4.*3.79080679921875e-6+cos(x_3).^4.*cos(x_4).^2.*6.757062187003037e-11+cos(x_3).^4.*cos(x_5).^2.*6.757062187003037e-11+cos(x_3).^4.*cos(x_6).^2.*6.757062187003037e-11+cos(x_3).^2.*sin(x_3).^2.*7.5816135984375e-6+cos(x_4).^2.*sin(x_3).^4.*6.757062187003037e-11+cos(x_5).^2.*sin(x_3).^4.*6.757062187003037e-11+cos(x_6).^2.*sin(x_3).^4.*6.757062187003037e-11+cos(x_3).^2.*cos(x_4).^2.*sin(x_3).^2.*1.351412437400607e-10+cos(x_3).^2.*cos(x_5).^2.*sin(x_3).^2.*1.351412437400607e-10+cos(x_3).^2.*cos(x_6).^2.*sin(x_3).^2.*1.351412437400607e-10)+(x_8.*x_9.*cos(x_3).^3.*cos(x_4).*sin(x_3).^2.*sin(x_4).*sin(x_6).^4.*2.620302164406908e-24)./(cos(x_3).^4.*3.79080679921875e-6+sin(x_3).^4.*3.79080679921875e-6+cos(x_3).^4.*cos(x_4).^2.*6.757062187003037e-11+cos(x_3).^4.*cos(x_5).^2.*6.757062187003037e-11+cos(x_3).^4.*cos(x_6).^2.*6.757062187003037e-11+cos(x_3).^2.*sin(x_3).^2.*7.5816135984375e-6+cos(x_4).^2.*sin(x_3).^4.*6.757062187003037e-11+cos(x_5).^2.*sin(x_3).^4.*6.757062187003037e-11+cos(x_6).^2.*sin(x_3).^4.*6.757062187003037e-11+cos(x_3).^2.*cos(x_4).^2.*sin(x_3).^2.*1.351412437400607e-10+cos(x_3).^2.*cos(x_5).^2.*sin(x_3).^2.*1.351412437400607e-10+cos(x_3).^2.*cos(x_6).^2.*sin(x_3).^2.*1.351412437400607e-10)+(x_8.*x_9.*cos(x_3).^3.*cos(x_5).*sin(x_3).^2.*sin(x_5).*sin(x_6).^2.*1.470104929075305e-19)./(cos(x_3).^4.*3.79080679921875e-6+sin(x_3).^4.*3.79080679921875e-6+cos(x_3).^4.*cos(x_4).^2.*6.757062187003037e-11+cos(x_3).^4.*cos(x_5).^2.*6.757062187003037e-11+cos(x_3).^4.*cos(x_6).^2.*6.757062187003037e-11+cos(x_3).^2.*sin(x_3).^2.*7.5816135984375e-6+cos(x_4).^2.*sin(x_3).^4.*6.757062187003037e-11+cos(x_5).^2.*sin(x_3).^4.*6.757062187003037e-11+cos(x_6).^2.*sin(x_3).^4.*6.757062187003037e-11+cos(x_3).^2.*cos(x_4).^2.*sin(x_3).^2.*1.351412437400607e-10+cos(x_3).^2.*cos(x_5).^2.*sin(x_3).^2.*1.351412437400607e-10+cos(x_3).^2.*cos(x_6).^2.*sin(x_3).^2.*1.351412437400607e-10)-(x_8.*x_9.*cos(x_3).^3.*cos(x_5).*sin(x_3).^2.*sin(x_4).^4.*sin(x_5).*1.310151082203454e-24)./(cos(x_3).^4.*3.79080679921875e-6+sin(x_3).^4.*3.79080679921875e-6+cos(x_3).^4.*cos(x_4).^2.*6.757062187003037e-11+cos(x_3).^4.*cos(x_5).^2.*6.757062187003037e-11+cos(x_3).^4.*cos(x_6).^2.*6.757062187003037e-11+cos(x_3).^2.*sin(x_3).^2.*7.5816135984375e-6+cos(x_4).^2.*sin(x_3).^4.*6.757062187003037e-11+cos(x_5).^2.*sin(x_3).^4.*6.757062187003037e-11+cos(x_6).^2.*sin(x_3).^4.*6.757062187003037e-11+cos(x_3).^2.*cos(x_4).^2.*sin(x_3).^2.*1.351412437400607e-10+cos(x_3).^2.*cos(x_5).^2.*sin(x_3).^2.*1.351412437400607e-10+cos(x_3).^2.*cos(x_6).^2.*sin(x_3).^2.*1.351412437400607e-10)+(x_8.*x_9.*cos(x_3).^3.*cos(x_6).*sin(x_3).^2.*sin(x_4).^2.*sin(x_6).*1.470104929075305e-19)./(cos(x_3).^4.*3.79080679921875e-6+sin(x_3).^4.*3.79080679921875e-6+cos(x_3).^4.*cos(x_4).^2.*6.757062187003037e-11+cos(x_3).^4.*cos(x_5).^2.*6.757062187003037e-11+cos(x_3).^4.*cos(x_6).^2.*6.757062187003037e-11+cos(x_3).^2.*sin(x_3).^2.*7.5816135984375e-6+cos(x_4).^2.*sin(x_3).^4.*6.757062187003037e-11+cos(x_5).^2.*sin(x_3).^4.*6.757062187003037e-11+cos(x_6).^2.*sin(x_3).^4.*6.757062187003037e-11+cos(x_3).^2.*cos(x_4).^2.*sin(x_3).^2.*1.351412437400607e-10+cos(x_3).^2.*cos(x_5).^2.*sin(x_3).^2.*1.351412437400607e-10+cos(x_3).^2.*cos(x_6).^2.*sin(x_3).^2.*1.351412437400607e-10)-(x_8.*x_9.*cos(x_3).^4.*cos(x_5).*sin(x_3).*sin(x_4).^2.*sin(x_5).^3.*2.269248239967731e-24)./(cos(x_3).^4.*3.79080679921875e-6+sin(x_3).^4.*3.79080679921875e-6+cos(x_3).^4.*cos(x_4).^2.*6.757062187003037e-11+cos(x_3).^4.*cos(x_5).^2.*6.757062187003037e-11+cos(x_3).^4.*cos(x_6).^2.*6.757062187003037e-11+cos(x_3).^2.*sin(x_3).^2.*7.5816135984375e-6+cos(x_4).^2.*sin(x_3).^4.*6.757062187003037e-11+cos(x_5).^2.*sin(x_3).^4.*6.757062187003037e-11+cos(x_6).^2.*sin(x_3).^4.*6.757062187003037e-11+cos(x_3).^2.*cos(x_4).^2.*sin(x_3).^2.*1.351412437400607e-10+cos(x_3).^2.*cos(x_5).^2.*sin(x_3).^2.*1.351412437400607e-10+cos(x_3).^2.*cos(x_6).^2.*sin(x_3).^2.*1.351412437400607e-10)-(x_7.*x_9.*cos(x_3).*cos(x_5).*sin(x_3).^4.*sin(x_5).^3.*sin(x_6).^2.*2.269248239967731e-24)./(cos(x_3).^4.*3.79080679921875e-6+sin(x_3).^4.*3.79080679921875e-6+cos(x_3).^4.*cos(x_4).^2.*6.757062187003037e-11+cos(x_3).^4.*cos(x_5).^2.*6.757062187003037e-11+cos(x_3).^4.*cos(x_6).^2.*6.757062187003037e-11+cos(x_3).^2.*sin(x_3).^2.*7.5816135984375e-6+cos(x_4).^2.*sin(x_3).^4.*6.757062187003037e-11+cos(x_5).^2.*sin(x_3).^4.*6.757062187003037e-11+cos(x_6).^2.*sin(x_3).^4.*6.757062187003037e-11+cos(x_3).^2.*cos(x_4).^2.*sin(x_3).^2.*1.351412437400607e-10+cos(x_3).^2.*cos(x_5).^2.*sin(x_3).^2.*1.351412437400607e-10+cos(x_3).^2.*cos(x_6).^2.*sin(x_3).^2.*1.351412437400607e-10)+(x_7.*x_9.*cos(x_3).*cos(x_6).*sin(x_3).^4.*sin(x_4).^2.*sin(x_6).^3.*2.269248239967731e-24)./(cos(x_3).^4.*3.79080679921875e-6+sin(x_3).^4.*3.79080679921875e-6+cos(x_3).^4.*cos(x_4).^2.*6.757062187003037e-11+cos(x_3).^4.*cos(x_5).^2.*6.757062187003037e-11+cos(x_3).^4.*cos(x_6).^2.*6.757062187003037e-11+cos(x_3).^2.*sin(x_3).^2.*7.5816135984375e-6+cos(x_4).^2.*sin(x_3).^4.*6.757062187003037e-11+cos(x_5).^2.*sin(x_3).^4.*6.757062187003037e-11+cos(x_6).^2.*sin(x_3).^4.*6.757062187003037e-11+cos(x_3).^2.*cos(x_4).^2.*sin(x_3).^2.*1.351412437400607e-10+cos(x_3).^2.*cos(x_5).^2.*sin(x_3).^2.*1.351412437400607e-10+cos(x_3).^2.*cos(x_6).^2.*sin(x_3).^2.*1.351412437400607e-10)+(x_7.*x_9.*cos(x_3).^2.*cos(x_5).*sin(x_3).^3.*sin(x_5).*sin(x_6).^4.*1.310151082203454e-24)./(cos(x_3).^4.*3.79080679921875e-6+sin(x_3).^4.*3.79080679921875e-6+cos(x_3).^4.*cos(x_4).^2.*6.757062187003037e-11+cos(x_3).^4.*cos(x_5).^2.*6.757062187003037e-11+cos(x_3).^4.*cos(x_6).^2.*6.757062187003037e-11+cos(x_3).^2.*sin(x_3).^2.*7.5816135984375e-6+cos(x_4).^2.*sin(x_3).^4.*6.757062187003037e-11+cos(x_5).^2.*sin(x_3).^4.*6.757062187003037e-11+cos(x_6).^2.*sin(x_3).^4.*6.757062187003037e-11+cos(x_3).^2.*cos(x_4).^2.*sin(x_3).^2.*1.351412437400607e-10+cos(x_3).^2.*cos(x_5).^2.*sin(x_3).^2.*1.351412437400607e-10+cos(x_3).^2.*cos(x_6).^2.*sin(x_3).^2.*1.351412437400607e-10)+(x_7.*x_9.*cos(x_3).^2.*cos(x_6).*sin(x_3).^3.*sin(x_4).^4.*sin(x_6).*1.310151082203454e-24)./(cos(x_3).^4.*3.79080679921875e-6+sin(x_3).^4.*3.79080679921875e-6+cos(x_3).^4.*cos(x_4).^2.*6.757062187003037e-11+cos(x_3).^4.*cos(x_5).^2.*6.757062187003037e-11+cos(x_3).^4.*cos(x_6).^2.*6.757062187003037e-11+cos(x_3).^2.*sin(x_3).^2.*7.5816135984375e-6+cos(x_4).^2.*sin(x_3).^4.*6.757062187003037e-11+cos(x_5).^2.*sin(x_3).^4.*6.757062187003037e-11+cos(x_6).^2.*sin(x_3).^4.*6.757062187003037e-11+cos(x_3).^2.*cos(x_4).^2.*sin(x_3).^2.*1.351412437400607e-10+cos(x_3).^2.*cos(x_5).^2.*sin(x_3).^2.*1.351412437400607e-10+cos(x_3).^2.*cos(x_6).^2.*sin(x_3).^2.*1.351412437400607e-10)-(x_7.*x_9.*cos(x_3).^3.*cos(x_5).*sin(x_3).^2.*sin(x_5).*sin(x_6).^4.*2.269248239967731e-24)./(cos(x_3).^4.*3.79080679921875e-6+sin(x_3).^4.*3.79080679921875e-6+cos(x_3).^4.*cos(x_4).^2.*6.757062187003037e-11+cos(x_3).^4.*cos(x_5).^2.*6.757062187003037e-11+cos(x_3).^4.*cos(x_6).^2.*6.757062187003037e-11+cos(x_3).^2.*sin(x_3).^2.*7.5816135984375e-6+cos(x_4).^2.*sin(x_3).^4.*6.757062187003037e-11+cos(x_5).^2.*sin(x_3).^4.*6.757062187003037e-11+cos(x_6).^2.*sin(x_3).^4.*6.757062187003037e-11+cos(x_3).^2.*cos(x_4).^2.*sin(x_3).^2.*1.351412437400607e-10+cos(x_3).^2.*cos(x_5).^2.*sin(x_3).^2.*1.351412437400607e-10+cos(x_3).^2.*cos(x_6).^2.*sin(x_3).^2.*1.351412437400607e-10)+(x_7.*x_9.*cos(x_3).^3.*cos(x_6).*sin(x_3).^2.*sin(x_4).^4.*sin(x_6).*2.269248239967731e-24)./(cos(x_3).^4.*3.79080679921875e-6+sin(x_3).^4.*3.79080679921875e-6+cos(x_3).^4.*cos(x_4).^2.*6.757062187003037e-11+cos(x_3).^4.*cos(x_5).^2.*6.757062187003037e-11+cos(x_3).^4.*cos(x_6).^2.*6.757062187003037e-11+cos(x_3).^2.*sin(x_3).^2.*7.5816135984375e-6+cos(x_4).^2.*sin(x_3).^4.*6.757062187003037e-11+cos(x_5).^2.*sin(x_3).^4.*6.757062187003037e-11+cos(x_6).^2.*sin(x_3).^4.*6.757062187003037e-11+cos(x_3).^2.*cos(x_4).^2.*sin(x_3).^2.*1.351412437400607e-10+cos(x_3).^2.*cos(x_5).^2.*sin(x_3).^2.*1.351412437400607e-10+cos(x_3).^2.*cos(x_6).^2.*sin(x_3).^2.*1.351412437400607e-10)+(x_7.*x_9.*cos(x_3).^4.*cos(x_5).*sin(x_3).*sin(x_5).^3.*sin(x_6).^2.*1.310151082203454e-24)./(cos(x_3).^4.*3.79080679921875e-6+sin(x_3).^4.*3.79080679921875e-6+cos(x_3).^4.*cos(x_4).^2.*6.757062187003037e-11+cos(x_3).^4.*cos(x_5).^2.*6.757062187003037e-11+cos(x_3).^4.*cos(x_6).^2.*6.757062187003037e-11+cos(x_3).^2.*sin(x_3).^2.*7.5816135984375e-6+cos(x_4).^2.*sin(x_3).^4.*6.757062187003037e-11+cos(x_5).^2.*sin(x_3).^4.*6.757062187003037e-11+cos(x_6).^2.*sin(x_3).^4.*6.757062187003037e-11+cos(x_3).^2.*cos(x_4).^2.*sin(x_3).^2.*1.351412437400607e-10+cos(x_3).^2.*cos(x_5).^2.*sin(x_3).^2.*1.351412437400607e-10+cos(x_3).^2.*cos(x_6).^2.*sin(x_3).^2.*1.351412437400607e-10)+(x_7.*x_9.*cos(x_3).^4.*cos(x_6).*sin(x_3).*sin(x_4).^2.*sin(x_6).^3.*1.310151082203454e-24)./(cos(x_3).^4.*3.79080679921875e-6+sin(x_3).^4.*3.79080679921875e-6+cos(x_3).^4.*cos(x_4).^2.*6.757062187003037e-11+cos(x_3).^4.*cos(x_5).^2.*6.757062187003037e-11+cos(x_3).^4.*cos(x_6).^2.*6.757062187003037e-11+cos(x_3).^2.*sin(x_3).^2.*7.5816135984375e-6+cos(x_4).^2.*sin(x_3).^4.*6.757062187003037e-11+cos(x_5).^2.*sin(x_3).^4.*6.757062187003037e-11+cos(x_6).^2.*sin(x_3).^4.*6.757062187003037e-11+cos(x_3).^2.*cos(x_4).^2.*sin(x_3).^2.*1.351412437400607e-10+cos(x_3).^2.*cos(x_5).^2.*sin(x_3).^2.*1.351412437400607e-10+cos(x_3).^2.*cos(x_6).^2.*sin(x_3).^2.*1.351412437400607e-10)-(x_8.*x_9.*cos(x_3).^2.*cos(x_6).*sin(x_3).^3.*sin(x_5).^2.*sin(x_6).*2.546296429615869e-19)./(cos(x_3).^4.*3.79080679921875e-6+sin(x_3).^4.*3.79080679921875e-6+cos(x_3).^4.*cos(x_4).^2.*6.757062187003037e-11+cos(x_3).^4.*cos(x_5).^2.*6.757062187003037e-11+cos(x_3).^4.*cos(x_6).^2.*6.757062187003037e-11+cos(x_3).^2.*sin(x_3).^2.*7.5816135984375e-6+cos(x_4).^2.*sin(x_3).^4.*6.757062187003037e-11+cos(x_5).^2.*sin(x_3).^4.*6.757062187003037e-11+cos(x_6).^2.*sin(x_3).^4.*6.757062187003037e-11+cos(x_3).^2.*cos(x_4).^2.*sin(x_3).^2.*1.351412437400607e-10+cos(x_3).^2.*cos(x_5).^2.*sin(x_3).^2.*1.351412437400607e-10+cos(x_3).^2.*cos(x_6).^2.*sin(x_3).^2.*1.351412437400607e-10)+(x_8.*x_9.*cos(x_3).^3.*cos(x_6).*sin(x_3).^2.*sin(x_5).^2.*sin(x_6).*1.470104929075305e-19)./(cos(x_3).^4.*3.79080679921875e-6+sin(x_3).^4.*3.79080679921875e-6+cos(x_3).^4.*cos(x_4).^2.*6.757062187003037e-11+cos(x_3).^4.*cos(x_5).^2.*6.757062187003037e-11+cos(x_3).^4.*cos(x_6).^2.*6.757062187003037e-11+cos(x_3).^2.*sin(x_3).^2.*7.5816135984375e-6+cos(x_4).^2.*sin(x_3).^4.*6.757062187003037e-11+cos(x_5).^2.*sin(x_3).^4.*6.757062187003037e-11+cos(x_6).^2.*sin(x_3).^4.*6.757062187003037e-11+cos(x_3).^2.*cos(x_4).^2.*sin(x_3).^2.*1.351412437400607e-10+cos(x_3).^2.*cos(x_5).^2.*sin(x_3).^2.*1.351412437400607e-10+cos(x_3).^2.*cos(x_6).^2.*sin(x_3).^2.*1.351412437400607e-10)+(x_7.*x_9.*cos(x_3).*cos(x_6).*sin(x_3).^4.*sin(x_5).^2.*sin(x_6).^3.*2.269248239967731e-24)./(cos(x_3).^4.*3.79080679921875e-6+sin(x_3).^4.*3.79080679921875e-6+cos(x_3).^4.*cos(x_4).^2.*6.757062187003037e-11+cos(x_3).^4.*cos(x_5).^2.*6.757062187003037e-11+cos(x_3).^4.*cos(x_6).^2.*6.757062187003037e-11+cos(x_3).^2.*sin(x_3).^2.*7.5816135984375e-6+cos(x_4).^2.*sin(x_3).^4.*6.757062187003037e-11+cos(x_5).^2.*sin(x_3).^4.*6.757062187003037e-11+cos(x_6).^2.*sin(x_3).^4.*6.757062187003037e-11+cos(x_3).^2.*cos(x_4).^2.*sin(x_3).^2.*1.351412437400607e-10+cos(x_3).^2.*cos(x_5).^2.*sin(x_3).^2.*1.351412437400607e-10+cos(x_3).^2.*cos(x_6).^2.*sin(x_3).^2.*1.351412437400607e-10)+(x_7.*x_9.*cos(x_3).^2.*cos(x_6).*sin(x_3).^3.*sin(x_5).^4.*sin(x_6).*1.310151082203454e-24)./(cos(x_3).^4.*3.79080679921875e-6+sin(x_3).^4.*3.79080679921875e-6+cos(x_3).^4.*cos(x_4).^2.*6.757062187003037e-11+cos(x_3).^4.*cos(x_5).^2.*6.757062187003037e-11+cos(x_3).^4.*cos(x_6).^2.*6.757062187003037e-11+cos(x_3).^2.*sin(x_3).^2.*7.5816135984375e-6+cos(x_4).^2.*sin(x_3).^4.*6.757062187003037e-11+cos(x_5).^2.*sin(x_3).^4.*6.757062187003037e-11+cos(x_6).^2.*sin(x_3).^4.*6.757062187003037e-11+cos(x_3).^2.*cos(x_4).^2.*sin(x_3).^2.*1.351412437400607e-10+cos(x_3).^2.*cos(x_5).^2.*sin(x_3).^2.*1.351412437400607e-10+cos(x_3).^2.*cos(x_6).^2.*sin(x_3).^2.*1.351412437400607e-10)+(x_7.*x_9.*cos(x_3).^3.*cos(x_6).*sin(x_3).^2.*sin(x_5).^4.*sin(x_6).*2.269248239967731e-24)./(cos(x_3).^4.*3.79080679921875e-6+sin(x_3).^4.*3.79080679921875e-6+cos(x_3).^4.*cos(x_4).^2.*6.757062187003037e-11+cos(x_3).^4.*cos(x_5).^2.*6.757062187003037e-11+cos(x_3).^4.*cos(x_6).^2.*6.757062187003037e-11+cos(x_3).^2.*sin(x_3).^2.*7.5816135984375e-6+cos(x_4).^2.*sin(x_3).^4.*6.757062187003037e-11+cos(x_5).^2.*sin(x_3).^4.*6.757062187003037e-11+cos(x_6).^2.*sin(x_3).^4.*6.757062187003037e-11+cos(x_3).^2.*cos(x_4).^2.*sin(x_3).^2.*1.351412437400607e-10+cos(x_3).^2.*cos(x_5).^2.*sin(x_3).^2.*1.351412437400607e-10+cos(x_3).^2.*cos(x_6).^2.*sin(x_3).^2.*1.351412437400607e-10)+(x_7.*x_9.*cos(x_3).^4.*cos(x_6).*sin(x_3).*sin(x_5).^2.*sin(x_6).^3.*1.310151082203454e-24)./(cos(x_3).^4.*3.79080679921875e-6+sin(x_3).^4.*3.79080679921875e-6+cos(x_3).^4.*cos(x_4).^2.*6.757062187003037e-11+cos(x_3).^4.*cos(x_5).^2.*6.757062187003037e-11+cos(x_3).^4.*cos(x_6).^2.*6.757062187003037e-11+cos(x_3).^2.*sin(x_3).^2.*7.5816135984375e-6+cos(x_4).^2.*sin(x_3).^4.*6.757062187003037e-11+cos(x_5).^2.*sin(x_3).^4.*6.757062187003037e-11+cos(x_6).^2.*sin(x_3).^4.*6.757062187003037e-11+cos(x_3).^2.*cos(x_4).^2.*sin(x_3).^2.*1.351412437400607e-10+cos(x_3).^2.*cos(x_5).^2.*sin(x_3).^2.*1.351412437400607e-10+cos(x_3).^2.*cos(x_6).^2.*sin(x_3).^2.*1.351412437400607e-10)-(x_7.*x_9.*cos(x_3).^5.*cos(x_5).*sin(x_4).^2.*sin(x_5).*sin(x_6).^2.*2.269248239967731e-24)./(cos(x_3).^4.*3.79080679921875e-6+sin(x_3).^4.*3.79080679921875e-6+cos(x_3).^4.*cos(x_4).^2.*6.757062187003037e-11+cos(x_3).^4.*cos(x_5).^2.*6.757062187003037e-11+cos(x_3).^4.*cos(x_6).^2.*6.757062187003037e-11+cos(x_3).^2.*sin(x_3).^2.*7.5816135984375e-6+cos(x_4).^2.*sin(x_3).^4.*6.757062187003037e-11+cos(x_5).^2.*sin(x_3).^4.*6.757062187003037e-11+cos(x_6).^2.*sin(x_3).^4.*6.757062187003037e-11+cos(x_3).^2.*cos(x_4).^2.*sin(x_3).^2.*1.351412437400607e-10+cos(x_3).^2.*cos(x_5).^2.*sin(x_3).^2.*1.351412437400607e-10+cos(x_3).^2.*cos(x_6).^2.*sin(x_3).^2.*1.351412437400607e-10)-(x_8.*x_9.*cos(x_3).*cos(x_5).*sin(x_3).^4.*sin(x_5).^3.*sin(x_6).^2.*1.310151082203454e-24)./(cos(x_3).^4.*3.79080679921875e-6+sin(x_3).^4.*3.79080679921875e-6+cos(x_3).^4.*cos(x_4).^2.*6.757062187003037e-11+cos(x_3).^4.*cos(x_5).^2.*6.757062187003037e-11+cos(x_3).^4.*cos(x_6).^2.*6.757062187003037e-11+cos(x_3).^2.*sin(x_3).^2.*7.5816135984375e-6+cos(x_4).^2.*sin(x_3).^4.*6.757062187003037e-11+cos(x_5).^2.*sin(x_3).^4.*6.757062187003037e-11+cos(x_6).^2.*sin(x_3).^4.*6.757062187003037e-11+cos(x_3).^2.*cos(x_4).^2.*sin(x_3).^2.*1.351412437400607e-10+cos(x_3).^2.*cos(x_5).^2.*sin(x_3).^2.*1.351412437400607e-10+cos(x_3).^2.*cos(x_6).^2.*sin(x_3).^2.*1.351412437400607e-10)-(x_8.*x_9.*cos(x_3).*cos(x_6).*sin(x_3).^4.*sin(x_4).^2.*sin(x_6).^3.*1.310151082203454e-24)./(cos(x_3).^4.*3.79080679921875e-6+sin(x_3).^4.*3.79080679921875e-6+cos(x_3).^4.*cos(x_4).^2.*6.757062187003037e-11+cos(x_3).^4.*cos(x_5).^2.*6.757062187003037e-11+cos(x_3).^4.*cos(x_6).^2.*6.757062187003037e-11+cos(x_3).^2.*sin(x_3).^2.*7.5816135984375e-6+cos(x_4).^2.*sin(x_3).^4.*6.757062187003037e-11+cos(x_5).^2.*sin(x_3).^4.*6.757062187003037e-11+cos(x_6).^2.*sin(x_3).^4.*6.757062187003037e-11+cos(x_3).^2.*cos(x_4).^2.*sin(x_3).^2.*1.351412437400607e-10+cos(x_3).^2.*cos(x_5).^2.*sin(x_3).^2.*1.351412437400607e-10+cos(x_3).^2.*cos(x_6).^2.*sin(x_3).^2.*1.351412437400607e-10)-(x_8.*x_9.*cos(x_3).^2.*cos(x_5).*sin(x_3).^3.*sin(x_5).*sin(x_6).^4.*2.269248239967731e-24)./(cos(x_3).^4.*3.79080679921875e-6+sin(x_3).^4.*3.79080679921875e-6+cos(x_3).^4.*cos(x_4).^2.*6.757062187003037e-11+cos(x_3).^4.*cos(x_5).^2.*6.757062187003037e-11+cos(x_3).^4.*cos(x_6).^2.*6.757062187003037e-11+cos(x_3).^2.*sin(x_3).^2.*7.5816135984375e-6+cos(x_4).^2.*sin(x_3).^4.*6.757062187003037e-11+cos(x_5).^2.*sin(x_3).^4.*6.757062187003037e-11+cos(x_6).^2.*sin(x_3).^4.*6.757062187003037e-11+cos(x_3).^2.*cos(x_4).^2.*sin(x_3).^2.*1.351412437400607e-10+cos(x_3).^2.*cos(x_5).^2.*sin(x_3).^2.*1.351412437400607e-10+cos(x_3).^2.*cos(x_6).^2.*sin(x_3).^2.*1.351412437400607e-10)+(x_8.*x_9.*cos(x_3).^2.*cos(x_6).*sin(x_3).^3.*sin(x_4).^4.*sin(x_6).*2.269248239967731e-24)./(cos(x_3).^4.*3.79080679921875e-6+sin(x_3).^4.*3.79080679921875e-6+cos(x_3).^4.*cos(x_4).^2.*6.757062187003037e-11+cos(x_3).^4.*cos(x_5).^2.*6.757062187003037e-11+cos(x_3).^4.*cos(x_6).^2.*6.757062187003037e-11+cos(x_3).^2.*sin(x_3).^2.*7.5816135984375e-6+cos(x_4).^2.*sin(x_3).^4.*6.757062187003037e-11+cos(x_5).^2.*sin(x_3).^4.*6.757062187003037e-11+cos(x_6).^2.*sin(x_3).^4.*6.757062187003037e-11+cos(x_3).^2.*cos(x_4).^2.*sin(x_3).^2.*1.351412437400607e-10+cos(x_3).^2.*cos(x_5).^2.*sin(x_3).^2.*1.351412437400607e-10+cos(x_3).^2.*cos(x_6).^2.*sin(x_3).^2.*1.351412437400607e-10)-(x_8.*x_9.*cos(x_3).^3.*cos(x_5).*sin(x_3).^2.*sin(x_5).*sin(x_6).^4.*1.310151082203454e-24)./(cos(x_3).^4.*3.79080679921875e-6+sin(x_3).^4.*3.79080679921875e-6+cos(x_3).^4.*cos(x_4).^2.*6.757062187003037e-11+cos(x_3).^4.*cos(x_5).^2.*6.757062187003037e-11+cos(x_3).^4.*cos(x_6).^2.*6.757062187003037e-11+cos(x_3).^2.*sin(x_3).^2.*7.5816135984375e-6+cos(x_4).^2.*sin(x_3).^4.*6.757062187003037e-11+cos(x_5).^2.*sin(x_3).^4.*6.757062187003037e-11+cos(x_6).^2.*sin(x_3).^4.*6.757062187003037e-11+cos(x_3).^2.*cos(x_4).^2.*sin(x_3).^2.*1.351412437400607e-10+cos(x_3).^2.*cos(x_5).^2.*sin(x_3).^2.*1.351412437400607e-10+cos(x_3).^2.*cos(x_6).^2.*sin(x_3).^2.*1.351412437400607e-10)-(x_8.*x_9.*cos(x_3).^3.*cos(x_6).*sin(x_3).^2.*sin(x_4).^4.*sin(x_6).*1.310151082203454e-24)./(cos(x_3).^4.*3.79080679921875e-6+sin(x_3).^4.*3.79080679921875e-6+cos(x_3).^4.*cos(x_4).^2.*6.757062187003037e-11+cos(x_3).^4.*cos(x_5).^2.*6.757062187003037e-11+cos(x_3).^4.*cos(x_6).^2.*6.757062187003037e-11+cos(x_3).^2.*sin(x_3).^2.*7.5816135984375e-6+cos(x_4).^2.*sin(x_3).^4.*6.757062187003037e-11+cos(x_5).^2.*sin(x_3).^4.*6.757062187003037e-11+cos(x_6).^2.*sin(x_3).^4.*6.757062187003037e-11+cos(x_3).^2.*cos(x_4).^2.*sin(x_3).^2.*1.351412437400607e-10+cos(x_3).^2.*cos(x_5).^2.*sin(x_3).^2.*1.351412437400607e-10+cos(x_3).^2.*cos(x_6).^2.*sin(x_3).^2.*1.351412437400607e-10)-(x_8.*x_9.*cos(x_3).^4.*cos(x_5).*sin(x_3).*sin(x_5).^3.*sin(x_6).^2.*2.269248239967731e-24)./(cos(x_3).^4.*3.79080679921875e-6+sin(x_3).^4.*3.79080679921875e-6+cos(x_3).^4.*cos(x_4).^2.*6.757062187003037e-11+cos(x_3).^4.*cos(x_5).^2.*6.757062187003037e-11+cos(x_3).^4.*cos(x_6).^2.*6.757062187003037e-11+cos(x_3).^2.*sin(x_3).^2.*7.5816135984375e-6+cos(x_4).^2.*sin(x_3).^4.*6.757062187003037e-11+cos(x_5).^2.*sin(x_3).^4.*6.757062187003037e-11+cos(x_6).^2.*sin(x_3).^4.*6.757062187003037e-11+cos(x_3).^2.*cos(x_4).^2.*sin(x_3).^2.*1.351412437400607e-10+cos(x_3).^2.*cos(x_5).^2.*sin(x_3).^2.*1.351412437400607e-10+cos(x_3).^2.*cos(x_6).^2.*sin(x_3).^2.*1.351412437400607e-10)+(x_8.*x_9.*cos(x_3).^4.*cos(x_6).*sin(x_3).*sin(x_4).^2.*sin(x_6).^3.*2.269248239967731e-24)./(cos(x_3).^4.*3.79080679921875e-6+sin(x_3).^4.*3.79080679921875e-6+cos(x_3).^4.*cos(x_4).^2.*6.757062187003037e-11+cos(x_3).^4.*cos(x_5).^2.*6.757062187003037e-11+cos(x_3).^4.*cos(x_6).^2.*6.757062187003037e-11+cos(x_3).^2.*sin(x_3).^2.*7.5816135984375e-6+cos(x_4).^2.*sin(x_3).^4.*6.757062187003037e-11+cos(x_5).^2.*sin(x_3).^4.*6.757062187003037e-11+cos(x_6).^2.*sin(x_3).^4.*6.757062187003037e-11+cos(x_3).^2.*cos(x_4).^2.*sin(x_3).^2.*1.351412437400607e-10+cos(x_3).^2.*cos(x_5).^2.*sin(x_3).^2.*1.351412437400607e-10+cos(x_3).^2.*cos(x_6).^2.*sin(x_3).^2.*1.351412437400607e-10)+(x_8.*x_9.*cos(x_3).^5.*cos(x_4).*sin(x_4).*sin(x_5).^2.*sin(x_6).^2.*2.620302164406908e-24)./(cos(x_3).^4.*3.79080679921875e-6+sin(x_3).^4.*3.79080679921875e-6+cos(x_3).^4.*cos(x_4).^2.*6.757062187003037e-11+cos(x_3).^4.*cos(x_5).^2.*6.757062187003037e-11+cos(x_3).^4.*cos(x_6).^2.*6.757062187003037e-11+cos(x_3).^2.*sin(x_3).^2.*7.5816135984375e-6+cos(x_4).^2.*sin(x_3).^4.*6.757062187003037e-11+cos(x_5).^2.*sin(x_3).^4.*6.757062187003037e-11+cos(x_6).^2.*sin(x_3).^4.*6.757062187003037e-11+cos(x_3).^2.*cos(x_4).^2.*sin(x_3).^2.*1.351412437400607e-10+cos(x_3).^2.*cos(x_5).^2.*sin(x_3).^2.*1.351412437400607e-10+cos(x_3).^2.*cos(x_6).^2.*sin(x_3).^2.*1.351412437400607e-10)+(x_7.*x_9.*cos(x_3).^5.*cos(x_6).*sin(x_4).^2.*sin(x_5).^2.*sin(x_6).*2.269248239967731e-24)./(cos(x_3).^4.*3.79080679921875e-6+sin(x_3).^4.*3.79080679921875e-6+cos(x_3).^4.*cos(x_4).^2.*6.757062187003037e-11+cos(x_3).^4.*cos(x_5).^2.*6.757062187003037e-11+cos(x_3).^4.*cos(x_6).^2.*6.757062187003037e-11+cos(x_3).^2.*sin(x_3).^2.*7.5816135984375e-6+cos(x_4).^2.*sin(x_3).^4.*6.757062187003037e-11+cos(x_5).^2.*sin(x_3).^4.*6.757062187003037e-11+cos(x_6).^2.*sin(x_3).^4.*6.757062187003037e-11+cos(x_3).^2.*cos(x_4).^2.*sin(x_3).^2.*1.351412437400607e-10+cos(x_3).^2.*cos(x_5).^2.*sin(x_3).^2.*1.351412437400607e-10+cos(x_3).^2.*cos(x_6).^2.*sin(x_3).^2.*1.351412437400607e-10)-(x_8.*x_9.*cos(x_3).*cos(x_6).*sin(x_3).^4.*sin(x_5).^2.*sin(x_6).^3.*1.310151082203454e-24)./(cos(x_3).^4.*3.79080679921875e-6+sin(x_3).^4.*3.79080679921875e-6+cos(x_3).^4.*cos(x_4).^2.*6.757062187003037e-11+cos(x_3).^4.*cos(x_5).^2.*6.757062187003037e-11+cos(x_3).^4.*cos(x_6).^2.*6.757062187003037e-11+cos(x_3).^2.*sin(x_3).^2.*7.5816135984375e-6+cos(x_4).^2.*sin(x_3).^4.*6.757062187003037e-11+cos(x_5).^2.*sin(x_3).^4.*6.757062187003037e-11+cos(x_6).^2.*sin(x_3).^4.*6.757062187003037e-11+cos(x_3).^2.*cos(x_4).^2.*sin(x_3).^2.*1.351412437400607e-10+cos(x_3).^2.*cos(x_5).^2.*sin(x_3).^2.*1.351412437400607e-10+cos(x_3).^2.*cos(x_6).^2.*sin(x_3).^2.*1.351412437400607e-10)+(x_8.*x_9.*cos(x_3).^2.*cos(x_6).*sin(x_3).^3.*sin(x_5).^4.*sin(x_6).*2.269248239967731e-24)./(cos(x_3).^4.*3.79080679921875e-6+sin(x_3).^4.*3.79080679921875e-6+cos(x_3).^4.*cos(x_4).^2.*6.757062187003037e-11+cos(x_3).^4.*cos(x_5).^2.*6.757062187003037e-11+cos(x_3).^4.*cos(x_6).^2.*6.757062187003037e-11+cos(x_3).^2.*sin(x_3).^2.*7.5816135984375e-6+cos(x_4).^2.*sin(x_3).^4.*6.757062187003037e-11+cos(x_5).^2.*sin(x_3).^4.*6.757062187003037e-11+cos(x_6).^2.*sin(x_3).^4.*6.757062187003037e-11+cos(x_3).^2.*cos(x_4).^2.*sin(x_3).^2.*1.351412437400607e-10+cos(x_3).^2.*cos(x_5).^2.*sin(x_3).^2.*1.351412437400607e-10+cos(x_3).^2.*cos(x_6).^2.*sin(x_3).^2.*1.351412437400607e-10)-(x_8.*x_9.*cos(x_3).^3.*cos(x_6).*sin(x_3).^2.*sin(x_5).^4.*sin(x_6).*1.310151082203454e-24)./(cos(x_3).^4.*3.79080679921875e-6+sin(x_3).^4.*3.79080679921875e-6+cos(x_3).^4.*cos(x_4).^2.*6.757062187003037e-11+cos(x_3).^4.*cos(x_5).^2.*6.757062187003037e-11+cos(x_3).^4.*cos(x_6).^2.*6.757062187003037e-11+cos(x_3).^2.*sin(x_3).^2.*7.5816135984375e-6+cos(x_4).^2.*sin(x_3).^4.*6.757062187003037e-11+cos(x_5).^2.*sin(x_3).^4.*6.757062187003037e-11+cos(x_6).^2.*sin(x_3).^4.*6.757062187003037e-11+cos(x_3).^2.*cos(x_4).^2.*sin(x_3).^2.*1.351412437400607e-10+cos(x_3).^2.*cos(x_5).^2.*sin(x_3).^2.*1.351412437400607e-10+cos(x_3).^2.*cos(x_6).^2.*sin(x_3).^2.*1.351412437400607e-10)+(x_8.*x_9.*cos(x_3).^4.*cos(x_6).*sin(x_3).*sin(x_5).^2.*sin(x_6).^3.*2.269248239967731e-24)./(cos(x_3).^4.*3.79080679921875e-6+sin(x_3).^4.*3.79080679921875e-6+cos(x_3).^4.*cos(x_4).^2.*6.757062187003037e-11+cos(x_3).^4.*cos(x_5).^2.*6.757062187003037e-11+cos(x_3).^4.*cos(x_6).^2.*6.757062187003037e-11+cos(x_3).^2.*sin(x_3).^2.*7.5816135984375e-6+cos(x_4).^2.*sin(x_3).^4.*6.757062187003037e-11+cos(x_5).^2.*sin(x_3).^4.*6.757062187003037e-11+cos(x_6).^2.*sin(x_3).^4.*6.757062187003037e-11+cos(x_3).^2.*cos(x_4).^2.*sin(x_3).^2.*1.351412437400607e-10+cos(x_3).^2.*cos(x_5).^2.*sin(x_3).^2.*1.351412437400607e-10+cos(x_3).^2.*cos(x_6).^2.*sin(x_3).^2.*1.351412437400607e-10)-(x_8.*x_9.*cos(x_3).^5.*cos(x_5).*sin(x_4).^2.*sin(x_5).*sin(x_6).^2.*1.310151082203454e-24)./(cos(x_3).^4.*3.79080679921875e-6+sin(x_3).^4.*3.79080679921875e-6+cos(x_3).^4.*cos(x_4).^2.*6.757062187003037e-11+cos(x_3).^4.*cos(x_5).^2.*6.757062187003037e-11+cos(x_3).^4.*cos(x_6).^2.*6.757062187003037e-11+cos(x_3).^2.*sin(x_3).^2.*7.5816135984375e-6+cos(x_4).^2.*sin(x_3).^4.*6.757062187003037e-11+cos(x_5).^2.*sin(x_3).^4.*6.757062187003037e-11+cos(x_6).^2.*sin(x_3).^4.*6.757062187003037e-11+cos(x_3).^2.*cos(x_4).^2.*sin(x_3).^2.*1.351412437400607e-10+cos(x_3).^2.*cos(x_5).^2.*sin(x_3).^2.*1.351412437400607e-10+cos(x_3).^2.*cos(x_6).^2.*sin(x_3).^2.*1.351412437400607e-10)-(x_8.*x_9.*cos(x_3).^5.*cos(x_6).*sin(x_4).^2.*sin(x_5).^2.*sin(x_6).*1.310151082203454e-24)./(cos(x_3).^4.*3.79080679921875e-6+sin(x_3).^4.*3.79080679921875e-6+cos(x_3).^4.*cos(x_4).^2.*6.757062187003037e-11+cos(x_3).^4.*cos(x_5).^2.*6.757062187003037e-11+cos(x_3).^4.*cos(x_6).^2.*6.757062187003037e-11+cos(x_3).^2.*sin(x_3).^2.*7.5816135984375e-6+cos(x_4).^2.*sin(x_3).^4.*6.757062187003037e-11+cos(x_5).^2.*sin(x_3).^4.*6.757062187003037e-11+cos(x_6).^2.*sin(x_3).^4.*6.757062187003037e-11+cos(x_3).^2.*cos(x_4).^2.*sin(x_3).^2.*1.351412437400607e-10+cos(x_3).^2.*cos(x_5).^2.*sin(x_3).^2.*1.351412437400607e-10+cos(x_3).^2.*cos(x_6).^2.*sin(x_3).^2.*1.351412437400607e-10)-(x_7.*x_9.*cos(x_3).^2.*cos(x_4).*sin(x_3).^2.*sin(x_4).*sin(x_5).^2.*1.607297550997493e-18)./(cos(x_3).^4.*1.5163227196875e-5+sin(x_3).^4.*1.5163227196875e-5+cos(x_3).^4.*cos(x_4).^2.*2.702824874801215e-10+cos(x_3).^4.*cos(x_5).^2.*2.702824874801215e-10+cos(x_3).^4.*cos(x_6).^2.*2.702824874801215e-10+cos(x_3).^2.*sin(x_3).^2.*3.032645439375e-5+cos(x_4).^2.*sin(x_3).^4.*2.702824874801215e-10+cos(x_5).^2.*sin(x_3).^4.*2.702824874801215e-10+cos(x_6).^2.*sin(x_3).^4.*2.702824874801215e-10+cos(x_3).^2.*cos(x_4).^2.*sin(x_3).^2.*5.40564974960243e-10+cos(x_3).^2.*cos(x_5).^2.*sin(x_3).^2.*5.40564974960243e-10+cos(x_3).^2.*cos(x_6).^2.*sin(x_3).^2.*5.40564974960243e-10)-(x_7.*x_9.*cos(x_3).^2.*cos(x_4).*sin(x_3).^2.*sin(x_4).*sin(x_6).^2.*1.607297550997493e-18)./(cos(x_3).^4.*1.5163227196875e-5+sin(x_3).^4.*1.5163227196875e-5+cos(x_3).^4.*cos(x_4).^2.*2.702824874801215e-10+cos(x_3).^4.*cos(x_5).^2.*2.702824874801215e-10+cos(x_3).^4.*cos(x_6).^2.*2.702824874801215e-10+cos(x_3).^2.*sin(x_3).^2.*3.032645439375e-5+cos(x_4).^2.*sin(x_3).^4.*2.702824874801215e-10+cos(x_5).^2.*sin(x_3).^4.*2.702824874801215e-10+cos(x_6).^2.*sin(x_3).^4.*2.702824874801215e-10+cos(x_3).^2.*cos(x_4).^2.*sin(x_3).^2.*5.40564974960243e-10+cos(x_3).^2.*cos(x_5).^2.*sin(x_3).^2.*5.40564974960243e-10+cos(x_3).^2.*cos(x_6).^2.*sin(x_3).^2.*5.40564974960243e-10)-(x_7.*x_9.*cos(x_3).^2.*cos(x_5).*sin(x_3).^2.*sin(x_4).^2.*sin(x_5).*4.39121857220618e-18)./(cos(x_3).^4.*1.5163227196875e-5+sin(x_3).^4.*1.5163227196875e-5+cos(x_3).^4.*cos(x_4).^2.*2.702824874801215e-10+cos(x_3).^4.*cos(x_5).^2.*2.702824874801215e-10+cos(x_3).^4.*cos(x_6).^2.*2.702824874801215e-10+cos(x_3).^2.*sin(x_3).^2.*3.032645439375e-5+cos(x_4).^2.*sin(x_3).^4.*2.702824874801215e-10+cos(x_5).^2.*sin(x_3).^4.*2.702824874801215e-10+cos(x_6).^2.*sin(x_3).^4.*2.702824874801215e-10+cos(x_3).^2.*cos(x_4).^2.*sin(x_3).^2.*5.40564974960243e-10+cos(x_3).^2.*cos(x_5).^2.*sin(x_3).^2.*5.40564974960243e-10+cos(x_3).^2.*cos(x_6).^2.*sin(x_3).^2.*5.40564974960243e-10)+(x_8.*x_9.*cos(x_3).^2.*cos(x_4).*sin(x_3).^2.*sin(x_4).*sin(x_5).^2.*5.998516123203674e-18)./(cos(x_3).^4.*1.5163227196875e-5+sin(x_3).^4.*1.5163227196875e-5+cos(x_3).^4.*cos(x_4).^2.*2.702824874801215e-10+cos(x_3).^4.*cos(x_5).^2.*2.702824874801215e-10+cos(x_3).^4.*cos(x_6).^2.*2.702824874801215e-10+cos(x_3).^2.*sin(x_3).^2.*3.032645439375e-5+cos(x_4).^2.*sin(x_3).^4.*2.702824874801215e-10+cos(x_5).^2.*sin(x_3).^4.*2.702824874801215e-10+cos(x_6).^2.*sin(x_3).^4.*2.702824874801215e-10+cos(x_3).^2.*cos(x_4).^2.*sin(x_3).^2.*5.40564974960243e-10+cos(x_3).^2.*cos(x_5).^2.*sin(x_3).^2.*5.40564974960243e-10+cos(x_3).^2.*cos(x_6).^2.*sin(x_3).^2.*5.40564974960243e-10)+(x_8.*x_9.*cos(x_3).^2.*cos(x_4).*sin(x_3).^2.*sin(x_4).*sin(x_6).^2.*5.998516123203674e-18)./(cos(x_3).^4.*1.5163227196875e-5+sin(x_3).^4.*1.5163227196875e-5+cos(x_3).^4.*cos(x_4).^2.*2.702824874801215e-10+cos(x_3).^4.*cos(x_5).^2.*2.702824874801215e-10+cos(x_3).^4.*cos(x_6).^2.*2.702824874801215e-10+cos(x_3).^2.*sin(x_3).^2.*3.032645439375e-5+cos(x_4).^2.*sin(x_3).^4.*2.702824874801215e-10+cos(x_5).^2.*sin(x_3).^4.*2.702824874801215e-10+cos(x_6).^2.*sin(x_3).^4.*2.702824874801215e-10+cos(x_3).^2.*cos(x_4).^2.*sin(x_3).^2.*5.40564974960243e-10+cos(x_3).^2.*cos(x_5).^2.*sin(x_3).^2.*5.40564974960243e-10+cos(x_3).^2.*cos(x_6).^2.*sin(x_3).^2.*5.40564974960243e-10)-(x_8.*x_9.*cos(x_3).^2.*cos(x_5).*sin(x_3).^2.*sin(x_4).^2.*sin(x_5).*4.39121857220618e-18)./(cos(x_3).^4.*1.5163227196875e-5+sin(x_3).^4.*1.5163227196875e-5+cos(x_3).^4.*cos(x_4).^2.*2.702824874801215e-10+cos(x_3).^4.*cos(x_5).^2.*2.702824874801215e-10+cos(x_3).^4.*cos(x_6).^2.*2.702824874801215e-10+cos(x_3).^2.*sin(x_3).^2.*3.032645439375e-5+cos(x_4).^2.*sin(x_3).^4.*2.702824874801215e-10+cos(x_5).^2.*sin(x_3).^4.*2.702824874801215e-10+cos(x_6).^2.*sin(x_3).^4.*2.702824874801215e-10+cos(x_3).^2.*cos(x_4).^2.*sin(x_3).^2.*5.40564974960243e-10+cos(x_3).^2.*cos(x_5).^2.*sin(x_3).^2.*5.40564974960243e-10+cos(x_3).^2.*cos(x_6).^2.*sin(x_3).^2.*5.40564974960243e-10)-(x_7.*x_9.*cos(x_3).^2.*cos(x_5).*sin(x_3).^2.*sin(x_5).*sin(x_6).^2.*4.39121857220618e-18)./(cos(x_3).^4.*1.5163227196875e-5+sin(x_3).^4.*1.5163227196875e-5+cos(x_3).^4.*cos(x_4).^2.*2.702824874801215e-10+cos(x_3).^4.*cos(x_5).^2.*2.702824874801215e-10+cos(x_3).^4.*cos(x_6).^2.*2.702824874801215e-10+cos(x_3).^2.*sin(x_3).^2.*3.032645439375e-5+cos(x_4).^2.*sin(x_3).^4.*2.702824874801215e-10+cos(x_5).^2.*sin(x_3).^4.*2.702824874801215e-10+cos(x_6).^2.*sin(x_3).^4.*2.702824874801215e-10+cos(x_3).^2.*cos(x_4).^2.*sin(x_3).^2.*5.40564974960243e-10+cos(x_3).^2.*cos(x_5).^2.*sin(x_3).^2.*5.40564974960243e-10+cos(x_3).^2.*cos(x_6).^2.*sin(x_3).^2.*5.40564974960243e-10)+(x_7.*x_9.*cos(x_3).^2.*cos(x_6).*sin(x_3).^2.*sin(x_4).^2.*sin(x_6).*5.998516123203674e-18)./(cos(x_3).^4.*1.5163227196875e-5+sin(x_3).^4.*1.5163227196875e-5+cos(x_3).^4.*cos(x_4).^2.*2.702824874801215e-10+cos(x_3).^4.*cos(x_5).^2.*2.702824874801215e-10+cos(x_3).^4.*cos(x_6).^2.*2.702824874801215e-10+cos(x_3).^2.*sin(x_3).^2.*3.032645439375e-5+cos(x_4).^2.*sin(x_3).^4.*2.702824874801215e-10+cos(x_5).^2.*sin(x_3).^4.*2.702824874801215e-10+cos(x_6).^2.*sin(x_3).^4.*2.702824874801215e-10+cos(x_3).^2.*cos(x_4).^2.*sin(x_3).^2.*5.40564974960243e-10+cos(x_3).^2.*cos(x_5).^2.*sin(x_3).^2.*5.40564974960243e-10+cos(x_3).^2.*cos(x_6).^2.*sin(x_3).^2.*5.40564974960243e-10)+(x_7.*x_9.*cos(x_3).^2.*cos(x_6).*sin(x_3).^2.*sin(x_5).^2.*sin(x_6).*5.998516123203674e-18)./(cos(x_3).^4.*1.5163227196875e-5+sin(x_3).^4.*1.5163227196875e-5+cos(x_3).^4.*cos(x_4).^2.*2.702824874801215e-10+cos(x_3).^4.*cos(x_5).^2.*2.702824874801215e-10+cos(x_3).^4.*cos(x_6).^2.*2.702824874801215e-10+cos(x_3).^2.*sin(x_3).^2.*3.032645439375e-5+cos(x_4).^2.*sin(x_3).^4.*2.702824874801215e-10+cos(x_5).^2.*sin(x_3).^4.*2.702824874801215e-10+cos(x_6).^2.*sin(x_3).^4.*2.702824874801215e-10+cos(x_3).^2.*cos(x_4).^2.*sin(x_3).^2.*5.40564974960243e-10+cos(x_3).^2.*cos(x_5).^2.*sin(x_3).^2.*5.40564974960243e-10+cos(x_3).^2.*cos(x_6).^2.*sin(x_3).^2.*5.40564974960243e-10)-(x_8.*x_9.*cos(x_3).^2.*cos(x_5).*sin(x_3).^2.*sin(x_5).*sin(x_6).^2.*4.39121857220618e-18)./(cos(x_3).^4.*1.5163227196875e-5+sin(x_3).^4.*1.5163227196875e-5+cos(x_3).^4.*cos(x_4).^2.*2.702824874801215e-10+cos(x_3).^4.*cos(x_5).^2.*2.702824874801215e-10+cos(x_3).^4.*cos(x_6).^2.*2.702824874801215e-10+cos(x_3).^2.*sin(x_3).^2.*3.032645439375e-5+cos(x_4).^2.*sin(x_3).^4.*2.702824874801215e-10+cos(x_5).^2.*sin(x_3).^4.*2.702824874801215e-10+cos(x_6).^2.*sin(x_3).^4.*2.702824874801215e-10+cos(x_3).^2.*cos(x_4).^2.*sin(x_3).^2.*5.40564974960243e-10+cos(x_3).^2.*cos(x_5).^2.*sin(x_3).^2.*5.40564974960243e-10+cos(x_3).^2.*cos(x_6).^2.*sin(x_3).^2.*5.40564974960243e-10)-(x_8.*x_9.*cos(x_3).^2.*cos(x_6).*sin(x_3).^2.*sin(x_4).^2.*sin(x_6).*1.607297550997493e-18)./(cos(x_3).^4.*1.5163227196875e-5+sin(x_3).^4.*1.5163227196875e-5+cos(x_3).^4.*cos(x_4).^2.*2.702824874801215e-10+cos(x_3).^4.*cos(x_5).^2.*2.702824874801215e-10+cos(x_3).^4.*cos(x_6).^2.*2.702824874801215e-10+cos(x_3).^2.*sin(x_3).^2.*3.032645439375e-5+cos(x_4).^2.*sin(x_3).^4.*2.702824874801215e-10+cos(x_5).^2.*sin(x_3).^4.*2.702824874801215e-10+cos(x_6).^2.*sin(x_3).^4.*2.702824874801215e-10+cos(x_3).^2.*cos(x_4).^2.*sin(x_3).^2.*5.40564974960243e-10+cos(x_3).^2.*cos(x_5).^2.*sin(x_3).^2.*5.40564974960243e-10+cos(x_3).^2.*cos(x_6).^2.*sin(x_3).^2.*5.40564974960243e-10)-(x_8.*x_9.*cos(x_3).^2.*cos(x_6).*sin(x_3).^2.*sin(x_5).^2.*sin(x_6).*1.607297550997493e-18)./(cos(x_3).^4.*1.5163227196875e-5+sin(x_3).^4.*1.5163227196875e-5+cos(x_3).^4.*cos(x_4).^2.*2.702824874801215e-10+cos(x_3).^4.*cos(x_5).^2.*2.702824874801215e-10+cos(x_3).^4.*cos(x_6).^2.*2.702824874801215e-10+cos(x_3).^2.*sin(x_3).^2.*3.032645439375e-5+cos(x_4).^2.*sin(x_3).^4.*2.702824874801215e-10+cos(x_5).^2.*sin(x_3).^4.*2.702824874801215e-10+cos(x_6).^2.*sin(x_3).^4.*2.702824874801215e-10+cos(x_3).^2.*cos(x_4).^2.*sin(x_3).^2.*5.40564974960243e-10+cos(x_3).^2.*cos(x_5).^2.*sin(x_3).^2.*5.40564974960243e-10+cos(x_3).^2.*cos(x_6).^2.*sin(x_3).^2.*5.40564974960243e-10)-(x_7.*x_9.*cos(x_4).*sin(x_3).^5.*sin(x_4).*sin(x_5).^2.*sin(x_6).^2.*2.620302164406908e-24)./(cos(x_3).^4.*3.79080679921875e-6+sin(x_3).^4.*3.79080679921875e-6+cos(x_3).^4.*cos(x_4).^2.*6.757062187003037e-11+cos(x_3).^4.*cos(x_5).^2.*6.757062187003037e-11+cos(x_3).^4.*cos(x_6).^2.*6.757062187003037e-11+cos(x_3).^2.*sin(x_3).^2.*7.5816135984375e-6+cos(x_4).^2.*sin(x_3).^4.*6.757062187003037e-11+cos(x_5).^2.*sin(x_3).^4.*6.757062187003037e-11+cos(x_6).^2.*sin(x_3).^4.*6.757062187003037e-11+cos(x_3).^2.*cos(x_4).^2.*sin(x_3).^2.*1.351412437400607e-10+cos(x_3).^2.*cos(x_5).^2.*sin(x_3).^2.*1.351412437400607e-10+cos(x_3).^2.*cos(x_6).^2.*sin(x_3).^2.*1.351412437400607e-10)+(x_7.*x_9.*cos(x_5).*sin(x_3).^5.*sin(x_4).^2.*sin(x_5).*sin(x_6).^2.*1.310151082203454e-24)./(cos(x_3).^4.*3.79080679921875e-6+sin(x_3).^4.*3.79080679921875e-6+cos(x_3).^4.*cos(x_4).^2.*6.757062187003037e-11+cos(x_3).^4.*cos(x_5).^2.*6.757062187003037e-11+cos(x_3).^4.*cos(x_6).^2.*6.757062187003037e-11+cos(x_3).^2.*sin(x_3).^2.*7.5816135984375e-6+cos(x_4).^2.*sin(x_3).^4.*6.757062187003037e-11+cos(x_5).^2.*sin(x_3).^4.*6.757062187003037e-11+cos(x_6).^2.*sin(x_3).^4.*6.757062187003037e-11+cos(x_3).^2.*cos(x_4).^2.*sin(x_3).^2.*1.351412437400607e-10+cos(x_3).^2.*cos(x_5).^2.*sin(x_3).^2.*1.351412437400607e-10+cos(x_3).^2.*cos(x_6).^2.*sin(x_3).^2.*1.351412437400607e-10)+(x_7.*x_9.*cos(x_6).*sin(x_3).^5.*sin(x_4).^2.*sin(x_5).^2.*sin(x_6).*1.310151082203454e-24)./(cos(x_3).^4.*3.79080679921875e-6+sin(x_3).^4.*3.79080679921875e-6+cos(x_3).^4.*cos(x_4).^2.*6.757062187003037e-11+cos(x_3).^4.*cos(x_5).^2.*6.757062187003037e-11+cos(x_3).^4.*cos(x_6).^2.*6.757062187003037e-11+cos(x_3).^2.*sin(x_3).^2.*7.5816135984375e-6+cos(x_4).^2.*sin(x_3).^4.*6.757062187003037e-11+cos(x_5).^2.*sin(x_3).^4.*6.757062187003037e-11+cos(x_6).^2.*sin(x_3).^4.*6.757062187003037e-11+cos(x_3).^2.*cos(x_4).^2.*sin(x_3).^2.*1.351412437400607e-10+cos(x_3).^2.*cos(x_5).^2.*sin(x_3).^2.*1.351412437400607e-10+cos(x_3).^2.*cos(x_6).^2.*sin(x_3).^2.*1.351412437400607e-10)-(x_8.*x_9.*cos(x_5).*sin(x_3).^5.*sin(x_4).^2.*sin(x_5).*sin(x_6).^2.*2.269248239967731e-24)./(cos(x_3).^4.*3.79080679921875e-6+sin(x_3).^4.*3.79080679921875e-6+cos(x_3).^4.*cos(x_4).^2.*6.757062187003037e-11+cos(x_3).^4.*cos(x_5).^2.*6.757062187003037e-11+cos(x_3).^4.*cos(x_6).^2.*6.757062187003037e-11+cos(x_3).^2.*sin(x_3).^2.*7.5816135984375e-6+cos(x_4).^2.*sin(x_3).^4.*6.757062187003037e-11+cos(x_5).^2.*sin(x_3).^4.*6.757062187003037e-11+cos(x_6).^2.*sin(x_3).^4.*6.757062187003037e-11+cos(x_3).^2.*cos(x_4).^2.*sin(x_3).^2.*1.351412437400607e-10+cos(x_3).^2.*cos(x_5).^2.*sin(x_3).^2.*1.351412437400607e-10+cos(x_3).^2.*cos(x_6).^2.*sin(x_3).^2.*1.351412437400607e-10)+(x_8.*x_9.*cos(x_6).*sin(x_3).^5.*sin(x_4).^2.*sin(x_5).^2.*sin(x_6).*2.269248239967731e-24)./(cos(x_3).^4.*3.79080679921875e-6+sin(x_3).^4.*3.79080679921875e-6+cos(x_3).^4.*cos(x_4).^2.*6.757062187003037e-11+cos(x_3).^4.*cos(x_5).^2.*6.757062187003037e-11+cos(x_3).^4.*cos(x_6).^2.*6.757062187003037e-11+cos(x_3).^2.*sin(x_3).^2.*7.5816135984375e-6+cos(x_4).^2.*sin(x_3).^4.*6.757062187003037e-11+cos(x_5).^2.*sin(x_3).^4.*6.757062187003037e-11+cos(x_6).^2.*sin(x_3).^4.*6.757062187003037e-11+cos(x_3).^2.*cos(x_4).^2.*sin(x_3).^2.*1.351412437400607e-10+cos(x_3).^2.*cos(x_5).^2.*sin(x_3).^2.*1.351412437400607e-10+cos(x_3).^2.*cos(x_6).^2.*sin(x_3).^2.*1.351412437400607e-10)-(x_7.*x_9.*cos(x_3).^2.*cos(x_4).*sin(x_3).^3.*sin(x_4).^3.*sin(x_5).^2.*5.240604328813817e-24)./(cos(x_3).^4.*3.79080679921875e-6+sin(x_3).^4.*3.79080679921875e-6+cos(x_3).^4.*cos(x_4).^2.*6.757062187003037e-11+cos(x_3).^4.*cos(x_5).^2.*6.757062187003037e-11+cos(x_3).^4.*cos(x_6).^2.*6.757062187003037e-11+cos(x_3).^2.*sin(x_3).^2.*7.5816135984375e-6+cos(x_4).^2.*sin(x_3).^4.*6.757062187003037e-11+cos(x_5).^2.*sin(x_3).^4.*6.757062187003037e-11+cos(x_6).^2.*sin(x_3).^4.*6.757062187003037e-11+cos(x_3).^2.*cos(x_4).^2.*sin(x_3).^2.*1.351412437400607e-10+cos(x_3).^2.*cos(x_5).^2.*sin(x_3).^2.*1.351412437400607e-10+cos(x_3).^2.*cos(x_6).^2.*sin(x_3).^2.*1.351412437400607e-10)-(x_7.*x_9.*cos(x_3).^2.*cos(x_4).*sin(x_3).^3.*sin(x_4).^3.*sin(x_6).^2.*5.240604328813817e-24)./(cos(x_3).^4.*3.79080679921875e-6+sin(x_3).^4.*3.79080679921875e-6+cos(x_3).^4.*cos(x_4).^2.*6.757062187003037e-11+cos(x_3).^4.*cos(x_5).^2.*6.757062187003037e-11+cos(x_3).^4.*cos(x_6).^2.*6.757062187003037e-11+cos(x_3).^2.*sin(x_3).^2.*7.5816135984375e-6+cos(x_4).^2.*sin(x_3).^4.*6.757062187003037e-11+cos(x_5).^2.*sin(x_3).^4.*6.757062187003037e-11+cos(x_6).^2.*sin(x_3).^4.*6.757062187003037e-11+cos(x_3).^2.*cos(x_4).^2.*sin(x_3).^2.*1.351412437400607e-10+cos(x_3).^2.*cos(x_5).^2.*sin(x_3).^2.*1.351412437400607e-10+cos(x_3).^2.*cos(x_6).^2.*sin(x_3).^2.*1.351412437400607e-10)+(x_7.*x_9.*cos(x_3).^2.*cos(x_5).*sin(x_3).^3.*sin(x_4).^2.*sin(x_5).^3.*2.620302164406908e-24)./(cos(x_3).^4.*3.79080679921875e-6+sin(x_3).^4.*3.79080679921875e-6+cos(x_3).^4.*cos(x_4).^2.*6.757062187003037e-11+cos(x_3).^4.*cos(x_5).^2.*6.757062187003037e-11+cos(x_3).^4.*cos(x_6).^2.*6.757062187003037e-11+cos(x_3).^2.*sin(x_3).^2.*7.5816135984375e-6+cos(x_4).^2.*sin(x_3).^4.*6.757062187003037e-11+cos(x_5).^2.*sin(x_3).^4.*6.757062187003037e-11+cos(x_6).^2.*sin(x_3).^4.*6.757062187003037e-11+cos(x_3).^2.*cos(x_4).^2.*sin(x_3).^2.*1.351412437400607e-10+cos(x_3).^2.*cos(x_5).^2.*sin(x_3).^2.*1.351412437400607e-10+cos(x_3).^2.*cos(x_6).^2.*sin(x_3).^2.*1.351412437400607e-10)-(x_7.*x_9.*cos(x_3).^3.*cos(x_5).*sin(x_3).^2.*sin(x_4).^2.*sin(x_5).^3.*4.538496479935463e-24)./(cos(x_3).^4.*3.79080679921875e-6+sin(x_3).^4.*3.79080679921875e-6+cos(x_3).^4.*cos(x_4).^2.*6.757062187003037e-11+cos(x_3).^4.*cos(x_5).^2.*6.757062187003037e-11+cos(x_3).^4.*cos(x_6).^2.*6.757062187003037e-11+cos(x_3).^2.*sin(x_3).^2.*7.5816135984375e-6+cos(x_4).^2.*sin(x_3).^4.*6.757062187003037e-11+cos(x_5).^2.*sin(x_3).^4.*6.757062187003037e-11+cos(x_6).^2.*sin(x_3).^4.*6.757062187003037e-11+cos(x_3).^2.*cos(x_4).^2.*sin(x_3).^2.*1.351412437400607e-10+cos(x_3).^2.*cos(x_5).^2.*sin(x_3).^2.*1.351412437400607e-10+cos(x_3).^2.*cos(x_6).^2.*sin(x_3).^2.*1.351412437400607e-10)+(x_8.*x_9.*cos(x_3).^3.*cos(x_4).*sin(x_3).^2.*sin(x_4).^3.*sin(x_5).^2.*5.240604328813817e-24)./(cos(x_3).^4.*3.79080679921875e-6+sin(x_3).^4.*3.79080679921875e-6+cos(x_3).^4.*cos(x_4).^2.*6.757062187003037e-11+cos(x_3).^4.*cos(x_5).^2.*6.757062187003037e-11+cos(x_3).^4.*cos(x_6).^2.*6.757062187003037e-11+cos(x_3).^2.*sin(x_3).^2.*7.5816135984375e-6+cos(x_4).^2.*sin(x_3).^4.*6.757062187003037e-11+cos(x_5).^2.*sin(x_3).^4.*6.757062187003037e-11+cos(x_6).^2.*sin(x_3).^4.*6.757062187003037e-11+cos(x_3).^2.*cos(x_4).^2.*sin(x_3).^2.*1.351412437400607e-10+cos(x_3).^2.*cos(x_5).^2.*sin(x_3).^2.*1.351412437400607e-10+cos(x_3).^2.*cos(x_6).^2.*sin(x_3).^2.*1.351412437400607e-10)-(x_8.*x_9.*cos(x_3).^2.*cos(x_5).*sin(x_3).^3.*sin(x_4).^2.*sin(x_5).^3.*4.538496479935463e-24)./(cos(x_3).^4.*3.79080679921875e-6+sin(x_3).^4.*3.79080679921875e-6+cos(x_3).^4.*cos(x_4).^2.*6.757062187003037e-11+cos(x_3).^4.*cos(x_5).^2.*6.757062187003037e-11+cos(x_3).^4.*cos(x_6).^2.*6.757062187003037e-11+cos(x_3).^2.*sin(x_3).^2.*7.5816135984375e-6+cos(x_4).^2.*sin(x_3).^4.*6.757062187003037e-11+cos(x_5).^2.*sin(x_3).^4.*6.757062187003037e-11+cos(x_6).^2.*sin(x_3).^4.*6.757062187003037e-11+cos(x_3).^2.*cos(x_4).^2.*sin(x_3).^2.*1.351412437400607e-10+cos(x_3).^2.*cos(x_5).^2.*sin(x_3).^2.*1.351412437400607e-10+cos(x_3).^2.*cos(x_6).^2.*sin(x_3).^2.*1.351412437400607e-10)+(x_8.*x_9.*cos(x_3).^3.*cos(x_4).*sin(x_3).^2.*sin(x_4).^3.*sin(x_6).^2.*5.240604328813817e-24)./(cos(x_3).^4.*3.79080679921875e-6+sin(x_3).^4.*3.79080679921875e-6+cos(x_3).^4.*cos(x_4).^2.*6.757062187003037e-11+cos(x_3).^4.*cos(x_5).^2.*6.757062187003037e-11+cos(x_3).^4.*cos(x_6).^2.*6.757062187003037e-11+cos(x_3).^2.*sin(x_3).^2.*7.5816135984375e-6+cos(x_4).^2.*sin(x_3).^4.*6.757062187003037e-11+cos(x_5).^2.*sin(x_3).^4.*6.757062187003037e-11+cos(x_6).^2.*sin(x_3).^4.*6.757062187003037e-11+cos(x_3).^2.*cos(x_4).^2.*sin(x_3).^2.*1.351412437400607e-10+cos(x_3).^2.*cos(x_5).^2.*sin(x_3).^2.*1.351412437400607e-10+cos(x_3).^2.*cos(x_6).^2.*sin(x_3).^2.*1.351412437400607e-10)-(x_8.*x_9.*cos(x_3).^3.*cos(x_5).*sin(x_3).^2.*sin(x_4).^2.*sin(x_5).^3.*2.620302164406908e-24)./(cos(x_3).^4.*3.79080679921875e-6+sin(x_3).^4.*3.79080679921875e-6+cos(x_3).^4.*cos(x_4).^2.*6.757062187003037e-11+cos(x_3).^4.*cos(x_5).^2.*6.757062187003037e-11+cos(x_3).^4.*cos(x_6).^2.*6.757062187003037e-11+cos(x_3).^2.*sin(x_3).^2.*7.5816135984375e-6+cos(x_4).^2.*sin(x_3).^4.*6.757062187003037e-11+cos(x_5).^2.*sin(x_3).^4.*6.757062187003037e-11+cos(x_6).^2.*sin(x_3).^4.*6.757062187003037e-11+cos(x_3).^2.*cos(x_4).^2.*sin(x_3).^2.*1.351412437400607e-10+cos(x_3).^2.*cos(x_5).^2.*sin(x_3).^2.*1.351412437400607e-10+cos(x_3).^2.*cos(x_6).^2.*sin(x_3).^2.*1.351412437400607e-10)+(x_7.*x_9.*cos(x_3).^2.*cos(x_5).*sin(x_3).^3.*sin(x_5).^3.*sin(x_6).^2.*2.620302164406908e-24)./(cos(x_3).^4.*3.79080679921875e-6+sin(x_3).^4.*3.79080679921875e-6+cos(x_3).^4.*cos(x_4).^2.*6.757062187003037e-11+cos(x_3).^4.*cos(x_5).^2.*6.757062187003037e-11+cos(x_3).^4.*cos(x_6).^2.*6.757062187003037e-11+cos(x_3).^2.*sin(x_3).^2.*7.5816135984375e-6+cos(x_4).^2.*sin(x_3).^4.*6.757062187003037e-11+cos(x_5).^2.*sin(x_3).^4.*6.757062187003037e-11+cos(x_6).^2.*sin(x_3).^4.*6.757062187003037e-11+cos(x_3).^2.*cos(x_4).^2.*sin(x_3).^2.*1.351412437400607e-10+cos(x_3).^2.*cos(x_5).^2.*sin(x_3).^2.*1.351412437400607e-10+cos(x_3).^2.*cos(x_6).^2.*sin(x_3).^2.*1.351412437400607e-10)+(x_7.*x_9.*cos(x_3).^2.*cos(x_6).*sin(x_3).^3.*sin(x_4).^2.*sin(x_6).^3.*2.620302164406908e-24)./(cos(x_3).^4.*3.79080679921875e-6+sin(x_3).^4.*3.79080679921875e-6+cos(x_3).^4.*cos(x_4).^2.*6.757062187003037e-11+cos(x_3).^4.*cos(x_5).^2.*6.757062187003037e-11+cos(x_3).^4.*cos(x_6).^2.*6.757062187003037e-11+cos(x_3).^2.*sin(x_3).^2.*7.5816135984375e-6+cos(x_4).^2.*sin(x_3).^4.*6.757062187003037e-11+cos(x_5).^2.*sin(x_3).^4.*6.757062187003037e-11+cos(x_6).^2.*sin(x_3).^4.*6.757062187003037e-11+cos(x_3).^2.*cos(x_4).^2.*sin(x_3).^2.*1.351412437400607e-10+cos(x_3).^2.*cos(x_5).^2.*sin(x_3).^2.*1.351412437400607e-10+cos(x_3).^2.*cos(x_6).^2.*sin(x_3).^2.*1.351412437400607e-10)-(x_7.*x_9.*cos(x_3).^3.*cos(x_5).*sin(x_3).^2.*sin(x_5).^3.*sin(x_6).^2.*4.538496479935463e-24)./(cos(x_3).^4.*3.79080679921875e-6+sin(x_3).^4.*3.79080679921875e-6+cos(x_3).^4.*cos(x_4).^2.*6.757062187003037e-11+cos(x_3).^4.*cos(x_5).^2.*6.757062187003037e-11+cos(x_3).^4.*cos(x_6).^2.*6.757062187003037e-11+cos(x_3).^2.*sin(x_3).^2.*7.5816135984375e-6+cos(x_4).^2.*sin(x_3).^4.*6.757062187003037e-11+cos(x_5).^2.*sin(x_3).^4.*6.757062187003037e-11+cos(x_6).^2.*sin(x_3).^4.*6.757062187003037e-11+cos(x_3).^2.*cos(x_4).^2.*sin(x_3).^2.*1.351412437400607e-10+cos(x_3).^2.*cos(x_5).^2.*sin(x_3).^2.*1.351412437400607e-10+cos(x_3).^2.*cos(x_6).^2.*sin(x_3).^2.*1.351412437400607e-10)+(x_7.*x_9.*cos(x_3).^3.*cos(x_6).*sin(x_3).^2.*sin(x_4).^2.*sin(x_6).^3.*4.538496479935463e-24)./(cos(x_3).^4.*3.79080679921875e-6+sin(x_3).^4.*3.79080679921875e-6+cos(x_3).^4.*cos(x_4).^2.*6.757062187003037e-11+cos(x_3).^4.*cos(x_5).^2.*6.757062187003037e-11+cos(x_3).^4.*cos(x_6).^2.*6.757062187003037e-11+cos(x_3).^2.*sin(x_3).^2.*7.5816135984375e-6+cos(x_4).^2.*sin(x_3).^4.*6.757062187003037e-11+cos(x_5).^2.*sin(x_3).^4.*6.757062187003037e-11+cos(x_6).^2.*sin(x_3).^4.*6.757062187003037e-11+cos(x_3).^2.*cos(x_4).^2.*sin(x_3).^2.*1.351412437400607e-10+cos(x_3).^2.*cos(x_5).^2.*sin(x_3).^2.*1.351412437400607e-10+cos(x_3).^2.*cos(x_6).^2.*sin(x_3).^2.*1.351412437400607e-10)+(x_7.*x_9.*cos(x_3).^2.*cos(x_6).*sin(x_3).^3.*sin(x_5).^2.*sin(x_6).^3.*2.620302164406908e-24)./(cos(x_3).^4.*3.79080679921875e-6+sin(x_3).^4.*3.79080679921875e-6+cos(x_3).^4.*cos(x_4).^2.*6.757062187003037e-11+cos(x_3).^4.*cos(x_5).^2.*6.757062187003037e-11+cos(x_3).^4.*cos(x_6).^2.*6.757062187003037e-11+cos(x_3).^2.*sin(x_3).^2.*7.5816135984375e-6+cos(x_4).^2.*sin(x_3).^4.*6.757062187003037e-11+cos(x_5).^2.*sin(x_3).^4.*6.757062187003037e-11+cos(x_6).^2.*sin(x_3).^4.*6.757062187003037e-11+cos(x_3).^2.*cos(x_4).^2.*sin(x_3).^2.*1.351412437400607e-10+cos(x_3).^2.*cos(x_5).^2.*sin(x_3).^2.*1.351412437400607e-10+cos(x_3).^2.*cos(x_6).^2.*sin(x_3).^2.*1.351412437400607e-10)+(x_7.*x_9.*cos(x_3).^3.*cos(x_6).*sin(x_3).^2.*sin(x_5).^2.*sin(x_6).^3.*4.538496479935463e-24)./(cos(x_3).^4.*3.79080679921875e-6+sin(x_3).^4.*3.79080679921875e-6+cos(x_3).^4.*cos(x_4).^2.*6.757062187003037e-11+cos(x_3).^4.*cos(x_5).^2.*6.757062187003037e-11+cos(x_3).^4.*cos(x_6).^2.*6.757062187003037e-11+cos(x_3).^2.*sin(x_3).^2.*7.5816135984375e-6+cos(x_4).^2.*sin(x_3).^4.*6.757062187003037e-11+cos(x_5).^2.*sin(x_3).^4.*6.757062187003037e-11+cos(x_6).^2.*sin(x_3).^4.*6.757062187003037e-11+cos(x_3).^2.*cos(x_4).^2.*sin(x_3).^2.*1.351412437400607e-10+cos(x_3).^2.*cos(x_5).^2.*sin(x_3).^2.*1.351412437400607e-10+cos(x_3).^2.*cos(x_6).^2.*sin(x_3).^2.*1.351412437400607e-10)-(x_8.*x_9.*cos(x_3).^2.*cos(x_5).*sin(x_3).^3.*sin(x_5).^3.*sin(x_6).^2.*4.538496479935463e-24)./(cos(x_3).^4.*3.79080679921875e-6+sin(x_3).^4.*3.79080679921875e-6+cos(x_3).^4.*cos(x_4).^2.*6.757062187003037e-11+cos(x_3).^4.*cos(x_5).^2.*6.757062187003037e-11+cos(x_3).^4.*cos(x_6).^2.*6.757062187003037e-11+cos(x_3).^2.*sin(x_3).^2.*7.5816135984375e-6+cos(x_4).^2.*sin(x_3).^4.*6.757062187003037e-11+cos(x_5).^2.*sin(x_3).^4.*6.757062187003037e-11+cos(x_6).^2.*sin(x_3).^4.*6.757062187003037e-11+cos(x_3).^2.*cos(x_4).^2.*sin(x_3).^2.*1.351412437400607e-10+cos(x_3).^2.*cos(x_5).^2.*sin(x_3).^2.*1.351412437400607e-10+cos(x_3).^2.*cos(x_6).^2.*sin(x_3).^2.*1.351412437400607e-10)+(x_8.*x_9.*cos(x_3).^2.*cos(x_6).*sin(x_3).^3.*sin(x_4).^2.*sin(x_6).^3.*4.538496479935463e-24)./(cos(x_3).^4.*3.79080679921875e-6+sin(x_3).^4.*3.79080679921875e-6+cos(x_3).^4.*cos(x_4).^2.*6.757062187003037e-11+cos(x_3).^4.*cos(x_5).^2.*6.757062187003037e-11+cos(x_3).^4.*cos(x_6).^2.*6.757062187003037e-11+cos(x_3).^2.*sin(x_3).^2.*7.5816135984375e-6+cos(x_4).^2.*sin(x_3).^4.*6.757062187003037e-11+cos(x_5).^2.*sin(x_3).^4.*6.757062187003037e-11+cos(x_6).^2.*sin(x_3).^4.*6.757062187003037e-11+cos(x_3).^2.*cos(x_4).^2.*sin(x_3).^2.*1.351412437400607e-10+cos(x_3).^2.*cos(x_5).^2.*sin(x_3).^2.*1.351412437400607e-10+cos(x_3).^2.*cos(x_6).^2.*sin(x_3).^2.*1.351412437400607e-10)-(x_8.*x_9.*cos(x_3).^3.*cos(x_5).*sin(x_3).^2.*sin(x_5).^3.*sin(x_6).^2.*2.620302164406908e-24)./(cos(x_3).^4.*3.79080679921875e-6+sin(x_3).^4.*3.79080679921875e-6+cos(x_3).^4.*cos(x_4).^2.*6.757062187003037e-11+cos(x_3).^4.*cos(x_5).^2.*6.757062187003037e-11+cos(x_3).^4.*cos(x_6).^2.*6.757062187003037e-11+cos(x_3).^2.*sin(x_3).^2.*7.5816135984375e-6+cos(x_4).^2.*sin(x_3).^4.*6.757062187003037e-11+cos(x_5).^2.*sin(x_3).^4.*6.757062187003037e-11+cos(x_6).^2.*sin(x_3).^4.*6.757062187003037e-11+cos(x_3).^2.*cos(x_4).^2.*sin(x_3).^2.*1.351412437400607e-10+cos(x_3).^2.*cos(x_5).^2.*sin(x_3).^2.*1.351412437400607e-10+cos(x_3).^2.*cos(x_6).^2.*sin(x_3).^2.*1.351412437400607e-10)-(x_8.*x_9.*cos(x_3).^3.*cos(x_6).*sin(x_3).^2.*sin(x_4).^2.*sin(x_6).^3.*2.620302164406908e-24)./(cos(x_3).^4.*3.79080679921875e-6+sin(x_3).^4.*3.79080679921875e-6+cos(x_3).^4.*cos(x_4).^2.*6.757062187003037e-11+cos(x_3).^4.*cos(x_5).^2.*6.757062187003037e-11+cos(x_3).^4.*cos(x_6).^2.*6.757062187003037e-11+cos(x_3).^2.*sin(x_3).^2.*7.5816135984375e-6+cos(x_4).^2.*sin(x_3).^4.*6.757062187003037e-11+cos(x_5).^2.*sin(x_3).^4.*6.757062187003037e-11+cos(x_6).^2.*sin(x_3).^4.*6.757062187003037e-11+cos(x_3).^2.*cos(x_4).^2.*sin(x_3).^2.*1.351412437400607e-10+cos(x_3).^2.*cos(x_5).^2.*sin(x_3).^2.*1.351412437400607e-10+cos(x_3).^2.*cos(x_6).^2.*sin(x_3).^2.*1.351412437400607e-10)+(x_8.*x_9.*cos(x_3).^2.*cos(x_6).*sin(x_3).^3.*sin(x_5).^2.*sin(x_6).^3.*4.538496479935463e-24)./(cos(x_3).^4.*3.79080679921875e-6+sin(x_3).^4.*3.79080679921875e-6+cos(x_3).^4.*cos(x_4).^2.*6.757062187003037e-11+cos(x_3).^4.*cos(x_5).^2.*6.757062187003037e-11+cos(x_3).^4.*cos(x_6).^2.*6.757062187003037e-11+cos(x_3).^2.*sin(x_3).^2.*7.5816135984375e-6+cos(x_4).^2.*sin(x_3).^4.*6.757062187003037e-11+cos(x_5).^2.*sin(x_3).^4.*6.757062187003037e-11+cos(x_6).^2.*sin(x_3).^4.*6.757062187003037e-11+cos(x_3).^2.*cos(x_4).^2.*sin(x_3).^2.*1.351412437400607e-10+cos(x_3).^2.*cos(x_5).^2.*sin(x_3).^2.*1.351412437400607e-10+cos(x_3).^2.*cos(x_6).^2.*sin(x_3).^2.*1.351412437400607e-10)-(x_8.*x_9.*cos(x_3).^3.*cos(x_6).*sin(x_3).^2.*sin(x_5).^2.*sin(x_6).^3.*2.620302164406908e-24)./(cos(x_3).^4.*3.79080679921875e-6+sin(x_3).^4.*3.79080679921875e-6+cos(x_3).^4.*cos(x_4).^2.*6.757062187003037e-11+cos(x_3).^4.*cos(x_5).^2.*6.757062187003037e-11+cos(x_3).^4.*cos(x_6).^2.*6.757062187003037e-11+cos(x_3).^2.*sin(x_3).^2.*7.5816135984375e-6+cos(x_4).^2.*sin(x_3).^4.*6.757062187003037e-11+cos(x_5).^2.*sin(x_3).^4.*6.757062187003037e-11+cos(x_6).^2.*sin(x_3).^4.*6.757062187003037e-11+cos(x_3).^2.*cos(x_4).^2.*sin(x_3).^2.*1.351412437400607e-10+cos(x_3).^2.*cos(x_5).^2.*sin(x_3).^2.*1.351412437400607e-10+cos(x_3).^2.*cos(x_6).^2.*sin(x_3).^2.*1.351412437400607e-10)-(x_7.*x_9.*cos(x_3).^4.*cos(x_4).*sin(x_3).*sin(x_4).*sin(x_5).^2.*sin(x_6).^2.*2.620302164406908e-24)./(cos(x_3).^4.*3.79080679921875e-6+sin(x_3).^4.*3.79080679921875e-6+cos(x_3).^4.*cos(x_4).^2.*6.757062187003037e-11+cos(x_3).^4.*cos(x_5).^2.*6.757062187003037e-11+cos(x_3).^4.*cos(x_6).^2.*6.757062187003037e-11+cos(x_3).^2.*sin(x_3).^2.*7.5816135984375e-6+cos(x_4).^2.*sin(x_3).^4.*6.757062187003037e-11+cos(x_5).^2.*sin(x_3).^4.*6.757062187003037e-11+cos(x_6).^2.*sin(x_3).^4.*6.757062187003037e-11+cos(x_3).^2.*cos(x_4).^2.*sin(x_3).^2.*1.351412437400607e-10+cos(x_3).^2.*cos(x_5).^2.*sin(x_3).^2.*1.351412437400607e-10+cos(x_3).^2.*cos(x_6).^2.*sin(x_3).^2.*1.351412437400607e-10)-(x_7.*x_9.*cos(x_3).*cos(x_5).*sin(x_3).^4.*sin(x_4).^2.*sin(x_5).*sin(x_6).^2.*2.269248239967731e-24)./(cos(x_3).^4.*3.79080679921875e-6+sin(x_3).^4.*3.79080679921875e-6+cos(x_3).^4.*cos(x_4).^2.*6.757062187003037e-11+cos(x_3).^4.*cos(x_5).^2.*6.757062187003037e-11+cos(x_3).^4.*cos(x_6).^2.*6.757062187003037e-11+cos(x_3).^2.*sin(x_3).^2.*7.5816135984375e-6+cos(x_4).^2.*sin(x_3).^4.*6.757062187003037e-11+cos(x_5).^2.*sin(x_3).^4.*6.757062187003037e-11+cos(x_6).^2.*sin(x_3).^4.*6.757062187003037e-11+cos(x_3).^2.*cos(x_4).^2.*sin(x_3).^2.*1.351412437400607e-10+cos(x_3).^2.*cos(x_5).^2.*sin(x_3).^2.*1.351412437400607e-10+cos(x_3).^2.*cos(x_6).^2.*sin(x_3).^2.*1.351412437400607e-10)+(x_7.*x_9.*cos(x_3).^4.*cos(x_5).*sin(x_3).*sin(x_4).^2.*sin(x_5).*sin(x_6).^2.*1.310151082203454e-24)./(cos(x_3).^4.*3.79080679921875e-6+sin(x_3).^4.*3.79080679921875e-6+cos(x_3).^4.*cos(x_4).^2.*6.757062187003037e-11+cos(x_3).^4.*cos(x_5).^2.*6.757062187003037e-11+cos(x_3).^4.*cos(x_6).^2.*6.757062187003037e-11+cos(x_3).^2.*sin(x_3).^2.*7.5816135984375e-6+cos(x_4).^2.*sin(x_3).^4.*6.757062187003037e-11+cos(x_5).^2.*sin(x_3).^4.*6.757062187003037e-11+cos(x_6).^2.*sin(x_3).^4.*6.757062187003037e-11+cos(x_3).^2.*cos(x_4).^2.*sin(x_3).^2.*1.351412437400607e-10+cos(x_3).^2.*cos(x_5).^2.*sin(x_3).^2.*1.351412437400607e-10+cos(x_3).^2.*cos(x_6).^2.*sin(x_3).^2.*1.351412437400607e-10)+(x_8.*x_9.*cos(x_3).*cos(x_4).*sin(x_3).^4.*sin(x_4).*sin(x_5).^2.*sin(x_6).^2.*2.620302164406908e-24)./(cos(x_3).^4.*3.79080679921875e-6+sin(x_3).^4.*3.79080679921875e-6+cos(x_3).^4.*cos(x_4).^2.*6.757062187003037e-11+cos(x_3).^4.*cos(x_5).^2.*6.757062187003037e-11+cos(x_3).^4.*cos(x_6).^2.*6.757062187003037e-11+cos(x_3).^2.*sin(x_3).^2.*7.5816135984375e-6+cos(x_4).^2.*sin(x_3).^4.*6.757062187003037e-11+cos(x_5).^2.*sin(x_3).^4.*6.757062187003037e-11+cos(x_6).^2.*sin(x_3).^4.*6.757062187003037e-11+cos(x_3).^2.*cos(x_4).^2.*sin(x_3).^2.*1.351412437400607e-10+cos(x_3).^2.*cos(x_5).^2.*sin(x_3).^2.*1.351412437400607e-10+cos(x_3).^2.*cos(x_6).^2.*sin(x_3).^2.*1.351412437400607e-10)+(x_7.*x_9.*cos(x_3).*cos(x_6).*sin(x_3).^4.*sin(x_4).^2.*sin(x_5).^2.*sin(x_6).*2.269248239967731e-24)./(cos(x_3).^4.*3.79080679921875e-6+sin(x_3).^4.*3.79080679921875e-6+cos(x_3).^4.*cos(x_4).^2.*6.757062187003037e-11+cos(x_3).^4.*cos(x_5).^2.*6.757062187003037e-11+cos(x_3).^4.*cos(x_6).^2.*6.757062187003037e-11+cos(x_3).^2.*sin(x_3).^2.*7.5816135984375e-6+cos(x_4).^2.*sin(x_3).^4.*6.757062187003037e-11+cos(x_5).^2.*sin(x_3).^4.*6.757062187003037e-11+cos(x_6).^2.*sin(x_3).^4.*6.757062187003037e-11+cos(x_3).^2.*cos(x_4).^2.*sin(x_3).^2.*1.351412437400607e-10+cos(x_3).^2.*cos(x_5).^2.*sin(x_3).^2.*1.351412437400607e-10+cos(x_3).^2.*cos(x_6).^2.*sin(x_3).^2.*1.351412437400607e-10)+(x_7.*x_9.*cos(x_3).^4.*cos(x_6).*sin(x_3).*sin(x_4).^2.*sin(x_5).^2.*sin(x_6).*1.310151082203454e-24)./(cos(x_3).^4.*3.79080679921875e-6+sin(x_3).^4.*3.79080679921875e-6+cos(x_3).^4.*cos(x_4).^2.*6.757062187003037e-11+cos(x_3).^4.*cos(x_5).^2.*6.757062187003037e-11+cos(x_3).^4.*cos(x_6).^2.*6.757062187003037e-11+cos(x_3).^2.*sin(x_3).^2.*7.5816135984375e-6+cos(x_4).^2.*sin(x_3).^4.*6.757062187003037e-11+cos(x_5).^2.*sin(x_3).^4.*6.757062187003037e-11+cos(x_6).^2.*sin(x_3).^4.*6.757062187003037e-11+cos(x_3).^2.*cos(x_4).^2.*sin(x_3).^2.*1.351412437400607e-10+cos(x_3).^2.*cos(x_5).^2.*sin(x_3).^2.*1.351412437400607e-10+cos(x_3).^2.*cos(x_6).^2.*sin(x_3).^2.*1.351412437400607e-10)-(x_8.*x_9.*cos(x_3).*cos(x_5).*sin(x_3).^4.*sin(x_4).^2.*sin(x_5).*sin(x_6).^2.*1.310151082203454e-24)./(cos(x_3).^4.*3.79080679921875e-6+sin(x_3).^4.*3.79080679921875e-6+cos(x_3).^4.*cos(x_4).^2.*6.757062187003037e-11+cos(x_3).^4.*cos(x_5).^2.*6.757062187003037e-11+cos(x_3).^4.*cos(x_6).^2.*6.757062187003037e-11+cos(x_3).^2.*sin(x_3).^2.*7.5816135984375e-6+cos(x_4).^2.*sin(x_3).^4.*6.757062187003037e-11+cos(x_5).^2.*sin(x_3).^4.*6.757062187003037e-11+cos(x_6).^2.*sin(x_3).^4.*6.757062187003037e-11+cos(x_3).^2.*cos(x_4).^2.*sin(x_3).^2.*1.351412437400607e-10+cos(x_3).^2.*cos(x_5).^2.*sin(x_3).^2.*1.351412437400607e-10+cos(x_3).^2.*cos(x_6).^2.*sin(x_3).^2.*1.351412437400607e-10)-(x_8.*x_9.*cos(x_3).^4.*cos(x_5).*sin(x_3).*sin(x_4).^2.*sin(x_5).*sin(x_6).^2.*2.269248239967731e-24)./(cos(x_3).^4.*3.79080679921875e-6+sin(x_3).^4.*3.79080679921875e-6+cos(x_3).^4.*cos(x_4).^2.*6.757062187003037e-11+cos(x_3).^4.*cos(x_5).^2.*6.757062187003037e-11+cos(x_3).^4.*cos(x_6).^2.*6.757062187003037e-11+cos(x_3).^2.*sin(x_3).^2.*7.5816135984375e-6+cos(x_4).^2.*sin(x_3).^4.*6.757062187003037e-11+cos(x_5).^2.*sin(x_3).^4.*6.757062187003037e-11+cos(x_6).^2.*sin(x_3).^4.*6.757062187003037e-11+cos(x_3).^2.*cos(x_4).^2.*sin(x_3).^2.*1.351412437400607e-10+cos(x_3).^2.*cos(x_5).^2.*sin(x_3).^2.*1.351412437400607e-10+cos(x_3).^2.*cos(x_6).^2.*sin(x_3).^2.*1.351412437400607e-10)-(x_8.*x_9.*cos(x_3).*cos(x_6).*sin(x_3).^4.*sin(x_4).^2.*sin(x_5).^2.*sin(x_6).*1.310151082203454e-24)./(cos(x_3).^4.*3.79080679921875e-6+sin(x_3).^4.*3.79080679921875e-6+cos(x_3).^4.*cos(x_4).^2.*6.757062187003037e-11+cos(x_3).^4.*cos(x_5).^2.*6.757062187003037e-11+cos(x_3).^4.*cos(x_6).^2.*6.757062187003037e-11+cos(x_3).^2.*sin(x_3).^2.*7.5816135984375e-6+cos(x_4).^2.*sin(x_3).^4.*6.757062187003037e-11+cos(x_5).^2.*sin(x_3).^4.*6.757062187003037e-11+cos(x_6).^2.*sin(x_3).^4.*6.757062187003037e-11+cos(x_3).^2.*cos(x_4).^2.*sin(x_3).^2.*1.351412437400607e-10+cos(x_3).^2.*cos(x_5).^2.*sin(x_3).^2.*1.351412437400607e-10+cos(x_3).^2.*cos(x_6).^2.*sin(x_3).^2.*1.351412437400607e-10)+(x_8.*x_9.*cos(x_3).^4.*cos(x_6).*sin(x_3).*sin(x_4).^2.*sin(x_5).^2.*sin(x_6).*2.269248239967731e-24)./(cos(x_3).^4.*3.79080679921875e-6+sin(x_3).^4.*3.79080679921875e-6+cos(x_3).^4.*cos(x_4).^2.*6.757062187003037e-11+cos(x_3).^4.*cos(x_5).^2.*6.757062187003037e-11+cos(x_3).^4.*cos(x_6).^2.*6.757062187003037e-11+cos(x_3).^2.*sin(x_3).^2.*7.5816135984375e-6+cos(x_4).^2.*sin(x_3).^4.*6.757062187003037e-11+cos(x_5).^2.*sin(x_3).^4.*6.757062187003037e-11+cos(x_6).^2.*sin(x_3).^4.*6.757062187003037e-11+cos(x_3).^2.*cos(x_4).^2.*sin(x_3).^2.*1.351412437400607e-10+cos(x_3).^2.*cos(x_5).^2.*sin(x_3).^2.*1.351412437400607e-10+cos(x_3).^2.*cos(x_6).^2.*sin(x_3).^2.*1.351412437400607e-10)-(x_7.*x_9.*cos(x_3).^2.*cos(x_4).*sin(x_3).^3.*sin(x_4).*sin(x_5).^2.*sin(x_6).^2.*5.240604328813817e-24)./(cos(x_3).^4.*3.79080679921875e-6+sin(x_3).^4.*3.79080679921875e-6+cos(x_3).^4.*cos(x_4).^2.*6.757062187003037e-11+cos(x_3).^4.*cos(x_5).^2.*6.757062187003037e-11+cos(x_3).^4.*cos(x_6).^2.*6.757062187003037e-11+cos(x_3).^2.*sin(x_3).^2.*7.5816135984375e-6+cos(x_4).^2.*sin(x_3).^4.*6.757062187003037e-11+cos(x_5).^2.*sin(x_3).^4.*6.757062187003037e-11+cos(x_6).^2.*sin(x_3).^4.*6.757062187003037e-11+cos(x_3).^2.*cos(x_4).^2.*sin(x_3).^2.*1.351412437400607e-10+cos(x_3).^2.*cos(x_5).^2.*sin(x_3).^2.*1.351412437400607e-10+cos(x_3).^2.*cos(x_6).^2.*sin(x_3).^2.*1.351412437400607e-10)+(x_7.*x_9.*cos(x_3).^2.*cos(x_5).*sin(x_3).^3.*sin(x_4).^2.*sin(x_5).*sin(x_6).^2.*2.620302164406908e-24)./(cos(x_3).^4.*3.79080679921875e-6+sin(x_3).^4.*3.79080679921875e-6+cos(x_3).^4.*cos(x_4).^2.*6.757062187003037e-11+cos(x_3).^4.*cos(x_5).^2.*6.757062187003037e-11+cos(x_3).^4.*cos(x_6).^2.*6.757062187003037e-11+cos(x_3).^2.*sin(x_3).^2.*7.5816135984375e-6+cos(x_4).^2.*sin(x_3).^4.*6.757062187003037e-11+cos(x_5).^2.*sin(x_3).^4.*6.757062187003037e-11+cos(x_6).^2.*sin(x_3).^4.*6.757062187003037e-11+cos(x_3).^2.*cos(x_4).^2.*sin(x_3).^2.*1.351412437400607e-10+cos(x_3).^2.*cos(x_5).^2.*sin(x_3).^2.*1.351412437400607e-10+cos(x_3).^2.*cos(x_6).^2.*sin(x_3).^2.*1.351412437400607e-10)-(x_7.*x_9.*cos(x_3).^3.*cos(x_5).*sin(x_3).^2.*sin(x_4).^2.*sin(x_5).*sin(x_6).^2.*4.538496479935463e-24)./(cos(x_3).^4.*3.79080679921875e-6+sin(x_3).^4.*3.79080679921875e-6+cos(x_3).^4.*cos(x_4).^2.*6.757062187003037e-11+cos(x_3).^4.*cos(x_5).^2.*6.757062187003037e-11+cos(x_3).^4.*cos(x_6).^2.*6.757062187003037e-11+cos(x_3).^2.*sin(x_3).^2.*7.5816135984375e-6+cos(x_4).^2.*sin(x_3).^4.*6.757062187003037e-11+cos(x_5).^2.*sin(x_3).^4.*6.757062187003037e-11+cos(x_6).^2.*sin(x_3).^4.*6.757062187003037e-11+cos(x_3).^2.*cos(x_4).^2.*sin(x_3).^2.*1.351412437400607e-10+cos(x_3).^2.*cos(x_5).^2.*sin(x_3).^2.*1.351412437400607e-10+cos(x_3).^2.*cos(x_6).^2.*sin(x_3).^2.*1.351412437400607e-10)+(x_8.*x_9.*cos(x_3).^3.*cos(x_4).*sin(x_3).^2.*sin(x_4).*sin(x_5).^2.*sin(x_6).^2.*5.240604328813817e-24)./(cos(x_3).^4.*3.79080679921875e-6+sin(x_3).^4.*3.79080679921875e-6+cos(x_3).^4.*cos(x_4).^2.*6.757062187003037e-11+cos(x_3).^4.*cos(x_5).^2.*6.757062187003037e-11+cos(x_3).^4.*cos(x_6).^2.*6.757062187003037e-11+cos(x_3).^2.*sin(x_3).^2.*7.5816135984375e-6+cos(x_4).^2.*sin(x_3).^4.*6.757062187003037e-11+cos(x_5).^2.*sin(x_3).^4.*6.757062187003037e-11+cos(x_6).^2.*sin(x_3).^4.*6.757062187003037e-11+cos(x_3).^2.*cos(x_4).^2.*sin(x_3).^2.*1.351412437400607e-10+cos(x_3).^2.*cos(x_5).^2.*sin(x_3).^2.*1.351412437400607e-10+cos(x_3).^2.*cos(x_6).^2.*sin(x_3).^2.*1.351412437400607e-10)+(x_7.*x_9.*cos(x_3).^2.*cos(x_6).*sin(x_3).^3.*sin(x_4).^2.*sin(x_5).^2.*sin(x_6).*2.620302164406908e-24)./(cos(x_3).^4.*3.79080679921875e-6+sin(x_3).^4.*3.79080679921875e-6+cos(x_3).^4.*cos(x_4).^2.*6.757062187003037e-11+cos(x_3).^4.*cos(x_5).^2.*6.757062187003037e-11+cos(x_3).^4.*cos(x_6).^2.*6.757062187003037e-11+cos(x_3).^2.*sin(x_3).^2.*7.5816135984375e-6+cos(x_4).^2.*sin(x_3).^4.*6.757062187003037e-11+cos(x_5).^2.*sin(x_3).^4.*6.757062187003037e-11+cos(x_6).^2.*sin(x_3).^4.*6.757062187003037e-11+cos(x_3).^2.*cos(x_4).^2.*sin(x_3).^2.*1.351412437400607e-10+cos(x_3).^2.*cos(x_5).^2.*sin(x_3).^2.*1.351412437400607e-10+cos(x_3).^2.*cos(x_6).^2.*sin(x_3).^2.*1.351412437400607e-10)+(x_7.*x_9.*cos(x_3).^3.*cos(x_6).*sin(x_3).^2.*sin(x_4).^2.*sin(x_5).^2.*sin(x_6).*4.538496479935463e-24)./(cos(x_3).^4.*3.79080679921875e-6+sin(x_3).^4.*3.79080679921875e-6+cos(x_3).^4.*cos(x_4).^2.*6.757062187003037e-11+cos(x_3).^4.*cos(x_5).^2.*6.757062187003037e-11+cos(x_3).^4.*cos(x_6).^2.*6.757062187003037e-11+cos(x_3).^2.*sin(x_3).^2.*7.5816135984375e-6+cos(x_4).^2.*sin(x_3).^4.*6.757062187003037e-11+cos(x_5).^2.*sin(x_3).^4.*6.757062187003037e-11+cos(x_6).^2.*sin(x_3).^4.*6.757062187003037e-11+cos(x_3).^2.*cos(x_4).^2.*sin(x_3).^2.*1.351412437400607e-10+cos(x_3).^2.*cos(x_5).^2.*sin(x_3).^2.*1.351412437400607e-10+cos(x_3).^2.*cos(x_6).^2.*sin(x_3).^2.*1.351412437400607e-10)-(x_8.*x_9.*cos(x_3).^2.*cos(x_5).*sin(x_3).^3.*sin(x_4).^2.*sin(x_5).*sin(x_6).^2.*4.538496479935463e-24)./(cos(x_3).^4.*3.79080679921875e-6+sin(x_3).^4.*3.79080679921875e-6+cos(x_3).^4.*cos(x_4).^2.*6.757062187003037e-11+cos(x_3).^4.*cos(x_5).^2.*6.757062187003037e-11+cos(x_3).^4.*cos(x_6).^2.*6.757062187003037e-11+cos(x_3).^2.*sin(x_3).^2.*7.5816135984375e-6+cos(x_4).^2.*sin(x_3).^4.*6.757062187003037e-11+cos(x_5).^2.*sin(x_3).^4.*6.757062187003037e-11+cos(x_6).^2.*sin(x_3).^4.*6.757062187003037e-11+cos(x_3).^2.*cos(x_4).^2.*sin(x_3).^2.*1.351412437400607e-10+cos(x_3).^2.*cos(x_5).^2.*sin(x_3).^2.*1.351412437400607e-10+cos(x_3).^2.*cos(x_6).^2.*sin(x_3).^2.*1.351412437400607e-10)-(x_8.*x_9.*cos(x_3).^3.*cos(x_5).*sin(x_3).^2.*sin(x_4).^2.*sin(x_5).*sin(x_6).^2.*2.620302164406908e-24)./(cos(x_3).^4.*3.79080679921875e-6+sin(x_3).^4.*3.79080679921875e-6+cos(x_3).^4.*cos(x_4).^2.*6.757062187003037e-11+cos(x_3).^4.*cos(x_5).^2.*6.757062187003037e-11+cos(x_3).^4.*cos(x_6).^2.*6.757062187003037e-11+cos(x_3).^2.*sin(x_3).^2.*7.5816135984375e-6+cos(x_4).^2.*sin(x_3).^4.*6.757062187003037e-11+cos(x_5).^2.*sin(x_3).^4.*6.757062187003037e-11+cos(x_6).^2.*sin(x_3).^4.*6.757062187003037e-11+cos(x_3).^2.*cos(x_4).^2.*sin(x_3).^2.*1.351412437400607e-10+cos(x_3).^2.*cos(x_5).^2.*sin(x_3).^2.*1.351412437400607e-10+cos(x_3).^2.*cos(x_6).^2.*sin(x_3).^2.*1.351412437400607e-10)+(x_8.*x_9.*cos(x_3).^2.*cos(x_6).*sin(x_3).^3.*sin(x_4).^2.*sin(x_5).^2.*sin(x_6).*4.538496479935463e-24)./(cos(x_3).^4.*3.79080679921875e-6+sin(x_3).^4.*3.79080679921875e-6+cos(x_3).^4.*cos(x_4).^2.*6.757062187003037e-11+cos(x_3).^4.*cos(x_5).^2.*6.757062187003037e-11+cos(x_3).^4.*cos(x_6).^2.*6.757062187003037e-11+cos(x_3).^2.*sin(x_3).^2.*7.5816135984375e-6+cos(x_4).^2.*sin(x_3).^4.*6.757062187003037e-11+cos(x_5).^2.*sin(x_3).^4.*6.757062187003037e-11+cos(x_6).^2.*sin(x_3).^4.*6.757062187003037e-11+cos(x_3).^2.*cos(x_4).^2.*sin(x_3).^2.*1.351412437400607e-10+cos(x_3).^2.*cos(x_5).^2.*sin(x_3).^2.*1.351412437400607e-10+cos(x_3).^2.*cos(x_6).^2.*sin(x_3).^2.*1.351412437400607e-10)-(x_8.*x_9.*cos(x_3).^3.*cos(x_6).*sin(x_3).^2.*sin(x_4).^2.*sin(x_5).^2.*sin(x_6).*2.620302164406908e-24)./(cos(x_3).^4.*3.79080679921875e-6+sin(x_3).^4.*3.79080679921875e-6+cos(x_3).^4.*cos(x_4).^2.*6.757062187003037e-11+cos(x_3).^4.*cos(x_5).^2.*6.757062187003037e-11+cos(x_3).^4.*cos(x_6).^2.*6.757062187003037e-11+cos(x_3).^2.*sin(x_3).^2.*7.5816135984375e-6+cos(x_4).^2.*sin(x_3).^4.*6.757062187003037e-11+cos(x_5).^2.*sin(x_3).^4.*6.757062187003037e-11+cos(x_6).^2.*sin(x_3).^4.*6.757062187003037e-11+cos(x_3).^2.*cos(x_4).^2.*sin(x_3).^2.*1.351412437400607e-10+cos(x_3).^2.*cos(x_5).^2.*sin(x_3).^2.*1.351412437400607e-10+cos(x_3).^2.*cos(x_6).^2.*sin(x_3).^2.*1.351412437400607e-10);